simulink model "Hospital"  (R2020b)
settings: Solver=VariableStepAuto  StartTime=0.0  StopTime=10.0  RelTol=1e-3
libraries: dspstat3 x5
(part 1 of 2)
settings Model: Creator=Stefano  LastModifiedBy=stefanopanzieri
settings SFSimCC: CustomCodeUndefinedFunction=UseInterfaceOnly

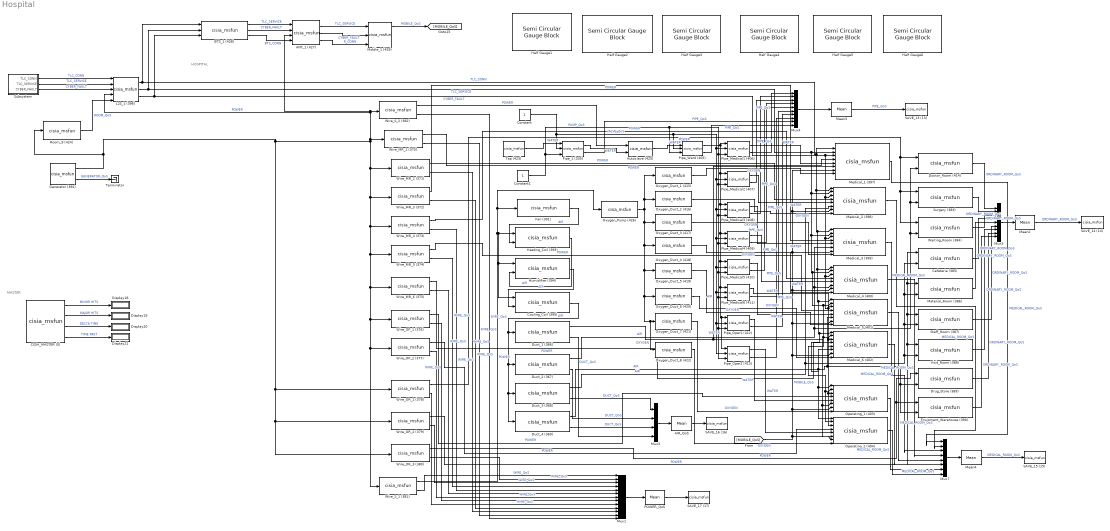
== system Hospital ==
  note: HOSPITAL
  note: MASTER
  AIR_QoS : dspstat3/Mean  run=off  InputProcessing=Columns as channels (frame based)  reset_popup=None  directionMode=Entire input  dimension=1  roiEnable=off  roiType=Rectangles  roiPortion=Entire ROI  roiOutput=Individual statistics for each ROI  roiFlag=off  roundingMode=Floor  overflowMode=off  outputDataTypeStr=Inherit: Same as accumulator  outputMin=[]  outputMax=[]  outputLastDataTypeStr=Inherit: Same as accumulator
  ANT_1 (427) : M-S-Function  FunctionName=cisia_msfun  Parameters=Parameter1, Parameter2, Parameter3, resources, Parameter10, codeupdate, step_received, step_computed, dynamic_computed, step_sended, id_entity, id_project, id_type, name_type, color  mask(S-function:msfcn_unit_delay){Parameter1='ANT_1', Parameter2=1, Parameter3='ORO', resources=, Parameter10=off, codeupdate=off, step_received=|, step_computed=, dynamic_computed=, step_sended=|, id_entity=427, id_project=6, id_type=55, name_type=CISCO_router, color=#EB7949}
      mask step_received=|
      | Connection=max(Connection_init,TLC_CONN);
      |
      | TLC_services=max(TLC_services_init,TLC_SERVICE);
      |
      |
      | Cyber_Fault=max(CYBER_FAULT, transpose([Dos_attack   MITM_attack  Port_Scan_Attack  Virus_Attack  BGP_hijacking]));
      |
      | % Vale 1 in presenza di fault
      | Conn_Fault=max([Dos_attack  Mechanical_Fault  1-POWER 1-ROOM_QoS] );
      |
      | Operative_Level=(1-Conn_Fault)*max(max(TLC_CONN),0.5);
      |
      |
      |
      | % Web Application Firewall and Enhanced application layer enrichment and protection
      mask step_sended=|
      | TLC_CONN=Connection*(1-Conn_Fault);
      | TLC_SERVICE=TLC_services*(1-Conn_Fault);
      | CYBER_FAULT=Cyber_Fault*(1-Conn_Fault);
      |
      | ROUTING_QoS=Operative_Level;
      mask prompts: Parameter1 "entity name"; Parameter2 "sampling time"; Parameter3 "project"; resources "input resources and state variables"; Parameter10 "Bring state variables to output"; codeupdate "update code from mask"
      mask help: This is a level-2 MATLAB file S-function which demonstrates CISIA entity
      mask DialogControl Container1 Prompt: All parameters
      mask Display: image('Icons/BTS_ANTENNA.png')
  Autoclave (425) : M-S-Function  FunctionName=cisia_msfun  Parameters=Parameter1, Parameter2, Parameter3, resources, Parameter10, codeupdate, step_received, step_computed, dynamic_computed, step_sended, id_entity, id_project, id_type, name_type, color  mask(S-function:msfcn_unit_delay){Parameter1='Autoclave', Parameter2=1, Parameter3='ORO', resources=, Parameter10=off, codeupdate=off, step_received=|, step_computed=, dynamic_computed=, step_sended=|, id_entity=425, id_project=6, id_type=33, name_type=Optical_Wire, color=#99CCFF}
      mask step_received=|
      | Connection=TLC_CONN;
      | TLC_services=TLC_SERVICE;
      | Cyber_Fault=CYBER_FAULT;
      |
      | Mechanical_Fault=max([Mechanical_Fault MECH_FAULT Mechanical_Fault_init]);
      |
      |
      | Operative_Level=1-Mechanical_Fault;
      mask step_sended=|
      | TLC_CONN=Connection*Operative_Level;
      | TLC_SERVICE=TLC_services*Operative_Level;
      | CYBER_FAULT=Cyber_Fault*Operative_Level;
      | MECH_FAULT=Mechanical_Fault;
      mask prompts: Parameter1 "entity name"; Parameter2 "sampling time"; Parameter3 "project"; resources "input resources and state variables"; Parameter10 "Bring state variables to output"; codeupdate "update code from mask"
      mask help: This is a level-2 MATLAB file S-function which demonstrates CISIA entity
      mask DialogControl Container1 Prompt: All parameters
      mask Display: disp('Autoclave')
  BTS_1 (428) : M-S-Function  FunctionName=cisia_msfun  Parameters=Parameter1, Parameter2, Parameter3, resources, Parameter10, codeupdate, step_received, step_computed, dynamic_computed, step_sended, id_entity, id_project, id_type, name_type, color  mask(S-function:msfcn_unit_delay){Parameter1='BTS_1', Parameter2=1, Parameter3='ORO', resources=, Parameter10=off, codeupdate=off, step_received=|, step_computed=, dynamic_computed=, step_sended=|, id_entity=428, id_project=6, id_type=54, name_type=CISCO_router, color=#EB7949}
      mask step_received=|
      | Connection=max(Connection_init,TLC_CONN);
      |
      | TLC_services=max(TLC_services_init,TLC_SERVICE);
      |
      |
      | Cyber_Fault=max(CYBER_FAULT, transpose([Dos_attack   MITM_attack  Port_Scan_Attack  Virus_Attack  BGP_hijacking]));
      |
      | % Vale 1 in presenza di fault
      | Conn_Fault=max([Dos_attack  Mechanical_Fault  1-POWER 1-ROOM_QoS] );
      |
      | Operative_Level=(1-Conn_Fault)*max(max(TLC_CONN),0.5);
      |
      |
      |
      | % Web Application Firewall and Enhanced application layer enrichment and protection
      mask step_sended=|
      | TLC_CONN=Connection*(1-Conn_Fault);
      | TLC_SERVICE=TLC_services*(1-Conn_Fault);
      | CYBER_FAULT=Cyber_Fault*(1-Conn_Fault);
      |
      | ROUTING_QoS=Operative_Level;
      mask prompts: Parameter1 "entity name"; Parameter2 "sampling time"; Parameter3 "project"; resources "input resources and state variables"; Parameter10 "Bring state variables to output"; codeupdate "update code from mask"
      mask help: This is a level-2 MATLAB file S-function which demonstrates CISIA entity
      mask DialogControl Container1 Prompt: All parameters
      mask Display: disp('BaseTransceiverStation')
  CISIA_MASTER (0) : M-S-Function  FunctionName=cisia_msfun  Parameters=Parameter1, Parameter2, Parameter3, resources, Parameter4, Parameter5, Parameter6, Parameter7, Parameter8, Parameter9  mask(S-function:msfcn_unit_delay){Parameter1='CISIA_MASTER', Parameter2=0.001, Parameter3='SistemiIoT', resources=off, Parameter4=on, Parameter5=off, Parameter6=off, Parameter7=off, Parameter8=1, Parameter9=off}
      mask prompts: Parameter1 "entity name"; Parameter2 "sampling time"; Parameter3 "project"; resources "Save status at each major hit"; Parameter4 "Show Operative Levels with colors"; Parameter5 "Load Entities from file"; Parameter6 "Load Start from Mask"; Parameter7 "Real Time"; Parameter8 "Real Time Hit (sec)"; Parameter9 "Skip saving"
      mask help: This is a level-2 MATLAB file S-function which demonstrates CISIA entity
      mask Display: disp('MASTER BLOCK')
  Cafeteria (385) : M-S-Function  FunctionName=cisia_msfun  Parameters=Parameter1, Parameter2, Parameter3, resources, Parameter10, codeupdate, step_received, step_computed, dynamic_computed, step_sended, id_entity, id_project, id_type, name_type, color  mask(S-function:msfcn_unit_delay){Parameter1='Cafeteria', Parameter2=1, Parameter3='ORO', resources=, Parameter10=off, codeupdate=off, step_received=|, step_computed=, dynamic_computed=, step_sended=|, id_entity=385, id_project=6, id_type=26, name_type=Optical_Wire, color=#99CCFF}
      mask step_received=|
      | Connection=TLC_CONN;
      | TLC_services=TLC_SERVICE;
      | Cyber_Fault=CYBER_FAULT;
      |
      | Mechanical_Fault=max([Mechanical_Fault MECH_FAULT Mechanical_Fault_init]);
      |
      |
      | Operative_Level=1-Mechanical_Fault;
      mask step_sended=|
      | TLC_CONN=Connection*Operative_Level;
      | TLC_SERVICE=TLC_services*Operative_Level;
      | CYBER_FAULT=Cyber_Fault*Operative_Level;
      | MECH_FAULT=Mechanical_Fault;
      mask prompts: Parameter1 "entity name"; Parameter2 "sampling time"; Parameter3 "project"; resources "input resources and state variables"; Parameter10 "Bring state variables to output"; codeupdate "update code from mask"
      mask help: This is a level-2 MATLAB file S-function which demonstrates CISIA entity
      mask DialogControl Container1 Prompt: All parameters
      mask Display: disp('Ordinary_Room')
  Constant : Constant
  Constant1 : Constant
  Cooling_Coil (395) : M-S-Function  FunctionName=cisia_msfun  Parameters=Parameter1, Parameter2, Parameter3, resources, Parameter10, codeupdate, step_received, step_computed, dynamic_computed, step_sended, id_entity, id_project, id_type, name_type, color  mask(S-function:msfcn_unit_delay){Parameter1='Cooling_Coil', Parameter2=1, Parameter3='ORO', resources=, Parameter10=off, codeupdate=off, step_received=|, step_computed=, dynamic_computed=, step_sended=|, id_entity=395, id_project=6, id_type=35, name_type=Optical_Wire, color=#99CCFF}
      mask step_received=|
      | Connection=TLC_CONN;
      | TLC_services=TLC_SERVICE;
      | Cyber_Fault=CYBER_FAULT;
      |
      | Mechanical_Fault=max([Mechanical_Fault MECH_FAULT Mechanical_Fault_init]);
      |
      |
      | Operative_Level=1-Mechanical_Fault;
      mask step_sended=|
      | TLC_CONN=Connection*Operative_Level;
      | TLC_SERVICE=TLC_services*Operative_Level;
      | CYBER_FAULT=Cyber_Fault*Operative_Level;
      | MECH_FAULT=Mechanical_Fault;
      mask prompts: Parameter1 "entity name"; Parameter2 "sampling time"; Parameter3 "project"; resources "input resources and state variables"; Parameter10 "Bring state variables to output"; codeupdate "update code from mask"
      mask help: This is a level-2 MATLAB file S-function which demonstrates CISIA entity
      mask DialogControl Container1 Prompt: All parameters
      mask Display: disp('Air_Conditioning_Element')
  Display{18..21} (4 alike) : Display
  Doctor_Room (414) : M-S-Function  FunctionName=cisia_msfun  Parameters=Parameter1, Parameter2, Parameter3, resources, Parameter10, codeupdate, step_received, step_computed, dynamic_computed, step_sended, id_entity, id_project, id_type, name_type, color  mask(S-function:msfcn_unit_delay){Parameter1='Doctor_Room', Parameter2=1, Parameter3='ORO', resources=, Parameter10=off, codeupdate=off, step_received=|, step_computed=, dynamic_computed=, step_sended=|, id_entity=414, id_project=6, id_type=26, name_type=Optical_Wire, color=#99CCFF}
      mask step_received=|
      | Connection=TLC_CONN;
      | TLC_services=TLC_SERVICE;
      | Cyber_Fault=CYBER_FAULT;
      |
      | Mechanical_Fault=max([Mechanical_Fault MECH_FAULT Mechanical_Fault_init]);
      |
      |
      | Operative_Level=1-Mechanical_Fault;
      mask step_sended=|
      | TLC_CONN=Connection*Operative_Level;
      | TLC_SERVICE=TLC_services*Operative_Level;
      | CYBER_FAULT=Cyber_Fault*Operative_Level;
      | MECH_FAULT=Mechanical_Fault;
      mask prompts: Parameter1 "entity name"; Parameter2 "sampling time"; Parameter3 "project"; resources "input resources and state variables"; Parameter10 "Bring state variables to output"; codeupdate "update code from mask"
      mask help: This is a level-2 MATLAB file S-function which demonstrates CISIA entity
      mask DialogControl Container1 Prompt: All parameters
      mask Display: disp('Ordinary_Room')
  Drug_Store (389) : M-S-Function  FunctionName=cisia_msfun  Parameters=Parameter1, Parameter2, Parameter3, resources, Parameter10, codeupdate, step_received, step_computed, dynamic_computed, step_sended, id_entity, id_project, id_type, name_type, color  mask(S-function:msfcn_unit_delay){Parameter1='Drug_Store', Parameter2=1, Parameter3='ORO', resources=, Parameter10=off, codeupdate=off, step_received=|, step_computed=, dynamic_computed=, step_sended=|, id_entity=389, id_project=6, id_type=26, name_type=Optical_Wire, color=#99CCFF}
      mask step_received=|
      | Connection=TLC_CONN;
      | TLC_services=TLC_SERVICE;
      | Cyber_Fault=CYBER_FAULT;
      |
      | Mechanical_Fault=max([Mechanical_Fault MECH_FAULT Mechanical_Fault_init]);
      |
      |
      | Operative_Level=1-Mechanical_Fault;
      mask step_sended=|
      | TLC_CONN=Connection*Operative_Level;
      | TLC_SERVICE=TLC_services*Operative_Level;
      | CYBER_FAULT=Cyber_Fault*Operative_Level;
      | MECH_FAULT=Mechanical_Fault;
      mask prompts: Parameter1 "entity name"; Parameter2 "sampling time"; Parameter3 "project"; resources "input resources and state variables"; Parameter10 "Bring state variables to output"; codeupdate "update code from mask"
      mask help: This is a level-2 MATLAB file S-function which demonstrates CISIA entity
      mask DialogControl Container1 Prompt: All parameters
      mask Display: disp('Ordinary_Room')
  Duct_1 (366) : M-S-Function  FunctionName=cisia_msfun  Parameters=Parameter1, Parameter2, Parameter3, resources, Parameter10, codeupdate, step_received, step_computed, dynamic_computed, step_sended, id_entity, id_project, id_type, name_type, color  mask(S-function:msfcn_unit_delay){Parameter1='Duct_1', Parameter2=1, Parameter3='ORO', resources=, Parameter10=off, codeupdate=off, step_received=|, step_computed=, dynamic_computed=, step_sended=|, id_entity=366, id_project=6, id_type=36, name_type=Optical_Wire, color=#99CCFF}
      mask step_received=|
      | Connection=TLC_CONN;
      | TLC_services=TLC_SERVICE;
      | Cyber_Fault=CYBER_FAULT;
      |
      | Mechanical_Fault=max([Mechanical_Fault MECH_FAULT Mechanical_Fault_init]);
      |
      |
      | Operative_Level=1-Mechanical_Fault;
      mask step_sended=|
      | TLC_CONN=Connection*Operative_Level;
      | TLC_SERVICE=TLC_services*Operative_Level;
      | CYBER_FAULT=Cyber_Fault*Operative_Level;
      | MECH_FAULT=Mechanical_Fault;
      mask prompts: Parameter1 "entity name"; Parameter2 "sampling time"; Parameter3 "project"; resources "input resources and state variables"; Parameter10 "Bring state variables to output"; codeupdate "update code from mask"
      mask help: This is a level-2 MATLAB file S-function which demonstrates CISIA entity
      mask DialogControl Container1 Prompt: All parameters
      mask Display: disp('Duct')
  Duct_2 (367) : M-S-Function  FunctionName=cisia_msfun  Parameters=Parameter1, Parameter2, Parameter3, resources, Parameter10, codeupdate, step_received, step_computed, dynamic_computed, step_sended, id_entity, id_project, id_type, name_type, color  mask(S-function:msfcn_unit_delay){Parameter1='Duct_2', Parameter2=1, Parameter3='ORO', resources=, Parameter10=off, codeupdate=off, step_received=|, step_computed=, dynamic_computed=, step_sended=|, id_entity=367, id_project=6, id_type=36, name_type=Optical_Wire, color=#99CCFF}
      mask step_received=|
      | Connection=TLC_CONN;
      | TLC_services=TLC_SERVICE;
      | Cyber_Fault=CYBER_FAULT;
      |
      | Mechanical_Fault=max([Mechanical_Fault MECH_FAULT Mechanical_Fault_init]);
      |
      |
      | Operative_Level=1-Mechanical_Fault;
      mask step_sended=|
      | TLC_CONN=Connection*Operative_Level;
      | TLC_SERVICE=TLC_services*Operative_Level;
      | CYBER_FAULT=Cyber_Fault*Operative_Level;
      | MECH_FAULT=Mechanical_Fault;
      mask prompts: Parameter1 "entity name"; Parameter2 "sampling time"; Parameter3 "project"; resources "input resources and state variables"; Parameter10 "Bring state variables to output"; codeupdate "update code from mask"
      mask help: This is a level-2 MATLAB file S-function which demonstrates CISIA entity
      mask DialogControl Container1 Prompt: All parameters
      mask Display: disp('Duct')
  Duct_3 (368) : M-S-Function  FunctionName=cisia_msfun  Parameters=Parameter1, Parameter2, Parameter3, resources, Parameter10, codeupdate, step_received, step_computed, dynamic_computed, step_sended, id_entity, id_project, id_type, name_type, color  mask(S-function:msfcn_unit_delay){Parameter1='Duct_3', Parameter2=1, Parameter3='ORO', resources=, Parameter10=off, codeupdate=off, step_received=|, step_computed=, dynamic_computed=, step_sended=|, id_entity=368, id_project=6, id_type=36, name_type=Optical_Wire, color=#99CCFF}
      mask step_received=|
      | Connection=TLC_CONN;
      | TLC_services=TLC_SERVICE;
      | Cyber_Fault=CYBER_FAULT;
      |
      | Mechanical_Fault=max([Mechanical_Fault MECH_FAULT Mechanical_Fault_init]);
      |
      |
      | Operative_Level=1-Mechanical_Fault;
      mask step_sended=|
      | TLC_CONN=Connection*Operative_Level;
      | TLC_SERVICE=TLC_services*Operative_Level;
      | CYBER_FAULT=Cyber_Fault*Operative_Level;
      | MECH_FAULT=Mechanical_Fault;
      mask prompts: Parameter1 "entity name"; Parameter2 "sampling time"; Parameter3 "project"; resources "input resources and state variables"; Parameter10 "Bring state variables to output"; codeupdate "update code from mask"
      mask help: This is a level-2 MATLAB file S-function which demonstrates CISIA entity
      mask DialogControl Container1 Prompt: All parameters
      mask Display: disp('Duct')
  Duct_4 (369) : M-S-Function  FunctionName=cisia_msfun  Parameters=Parameter1, Parameter2, Parameter3, resources, Parameter10, codeupdate, step_received, step_computed, dynamic_computed, step_sended, id_entity, id_project, id_type, name_type, color  mask(S-function:msfcn_unit_delay){Parameter1='Duct_4', Parameter2=1, Parameter3='ORO', resources=, Parameter10=off, codeupdate=off, step_received=|, step_computed=, dynamic_computed=, step_sended=|, id_entity=369, id_project=6, id_type=36, name_type=Optical_Wire, color=#99CCFF}
      mask step_received=|
      | Connection=TLC_CONN;
      | TLC_services=TLC_SERVICE;
      | Cyber_Fault=CYBER_FAULT;
      |
      | Mechanical_Fault=max([Mechanical_Fault MECH_FAULT Mechanical_Fault_init]);
      |
      |
      | Operative_Level=1-Mechanical_Fault;
      mask step_sended=|
      | TLC_CONN=Connection*Operative_Level;
      | TLC_SERVICE=TLC_services*Operative_Level;
      | CYBER_FAULT=Cyber_Fault*Operative_Level;
      | MECH_FAULT=Mechanical_Fault;
      mask prompts: Parameter1 "entity name"; Parameter2 "sampling time"; Parameter3 "project"; resources "input resources and state variables"; Parameter10 "Bring state variables to output"; codeupdate "update code from mask"
      mask help: This is a level-2 MATLAB file S-function which demonstrates CISIA entity
      mask DialogControl Container1 Prompt: All parameters
      mask Display: disp('Duct')
  Equipment_Warehouse (390) : M-S-Function  FunctionName=cisia_msfun  Parameters=Parameter1, Parameter2, Parameter3, resources, Parameter10, codeupdate, step_received, step_computed, dynamic_computed, step_sended, id_entity, id_project, id_type, name_type, color  mask(S-function:msfcn_unit_delay){Parameter1='Equipment_Warehouse', Parameter2=1, Parameter3='ORO', resources=, Parameter10=off, codeupdate=off, step_received=|, step_computed=, dynamic_computed=, step_sended=|, id_entity=390, id_project=6, id_type=26, name_type=Optical_Wire, color=#99CCFF}
      mask step_received=|
      | Connection=TLC_CONN;
      | TLC_services=TLC_SERVICE;
      | Cyber_Fault=CYBER_FAULT;
      |
      | Mechanical_Fault=max([Mechanical_Fault MECH_FAULT Mechanical_Fault_init]);
      |
      |
      | Operative_Level=1-Mechanical_Fault;
      mask step_sended=|
      | TLC_CONN=Connection*Operative_Level;
      | TLC_SERVICE=TLC_services*Operative_Level;
      | CYBER_FAULT=Cyber_Fault*Operative_Level;
      | MECH_FAULT=Mechanical_Fault;
      mask prompts: Parameter1 "entity name"; Parameter2 "sampling time"; Parameter3 "project"; resources "input resources and state variables"; Parameter10 "Bring state variables to output"; codeupdate "update code from mask"
      mask help: This is a level-2 MATLAB file S-function which demonstrates CISIA entity
      mask DialogControl Container1 Prompt: All parameters
      mask Display: disp('Ordinary_Room')
  Fan (391) : M-S-Function  FunctionName=cisia_msfun  Parameters=Parameter1, Parameter2, Parameter3, resources, Parameter10, codeupdate, step_received, step_computed, dynamic_computed, step_sended, id_entity, id_project, id_type, name_type, color  mask(S-function:msfcn_unit_delay){Parameter1='Fan', Parameter2=1, Parameter3='ORO', resources=, Parameter10=off, codeupdate=off, step_received=|, step_computed=, dynamic_computed=, step_sended=|, id_entity=391, id_project=6, id_type=34, name_type=Optical_Wire, color=#99CCFF}
      mask step_received=|
      | Connection=TLC_CONN;
      | TLC_services=TLC_SERVICE;
      | Cyber_Fault=CYBER_FAULT;
      |
      | Mechanical_Fault=max([Mechanical_Fault MECH_FAULT Mechanical_Fault_init]);
      |
      |
      | Operative_Level=1-Mechanical_Fault;
      mask step_sended=|
      | TLC_CONN=Connection*Operative_Level;
      | TLC_SERVICE=TLC_services*Operative_Level;
      | CYBER_FAULT=Cyber_Fault*Operative_Level;
      | MECH_FAULT=Mechanical_Fault;
      mask prompts: Parameter1 "entity name"; Parameter2 "sampling time"; Parameter3 "project"; resources "input resources and state variables"; Parameter10 "Bring state variables to output"; codeupdate "update code from mask"
      mask help: This is a level-2 MATLAB file S-function which demonstrates CISIA entity
      mask DialogControl Container1 Prompt: All parameters
      mask Display: disp('Fan')
  Generator (392) : M-S-Function  FunctionName=cisia_msfun  Parameters=Parameter1, Parameter2, Parameter3, resources, Parameter10, codeupdate, step_received, step_computed, dynamic_computed, step_sended, id_entity, id_project, id_type, name_type, color  mask(S-function:msfcn_unit_delay){Parameter1='Generator', Parameter2=1, Parameter3='ORO', resources=, Parameter10=off, codeupdate=off, step_received=|, step_computed=, dynamic_computed=, step_sended=|, id_entity=392, id_project=6, id_type=27, name_type=Optical_Wire, color=#99CCFF}
      mask step_received=|
      | Connection=TLC_CONN;
      | TLC_services=TLC_SERVICE;
      | Cyber_Fault=CYBER_FAULT;
      |
      | Mechanical_Fault=max([Mechanical_Fault MECH_FAULT Mechanical_Fault_init]);
      |
      |
      | Operative_Level=1-Mechanical_Fault;
      mask step_sended=|
      | TLC_CONN=Connection*Operative_Level;
      | TLC_SERVICE=TLC_services*Operative_Level;
      | CYBER_FAULT=Cyber_Fault*Operative_Level;
      | MECH_FAULT=Mechanical_Fault;
      mask prompts: Parameter1 "entity name"; Parameter2 "sampling time"; Parameter3 "project"; resources "input resources and state variables"; Parameter10 "Bring state variables to output"; codeupdate "update code from mask"
      mask help: This is a level-2 MATLAB file S-function which demonstrates CISIA entity
      mask DialogControl Container1 Prompt: All parameters
      mask Display: disp('Generator')
  Half Gauge{1..6} (6 alike) : SemiCircularGaugeBlock  ScaleMax=1
  Heating_Coil (393) : M-S-Function  FunctionName=cisia_msfun  Parameters=Parameter1, Parameter2, Parameter3, resources, Parameter10, codeupdate, step_received, step_computed, dynamic_computed, step_sended, id_entity, id_project, id_type, name_type, color  mask(S-function:msfcn_unit_delay){Parameter1='Heating_Coil', Parameter2=1, Parameter3='ORO', resources=, Parameter10=off, codeupdate=off, step_received=|, step_computed=, dynamic_computed=, step_sended=|, id_entity=393, id_project=6, id_type=35, name_type=Optical_Wire, color=#99CCFF}
      mask step_received=|
      | Connection=TLC_CONN;
      | TLC_services=TLC_SERVICE;
      | Cyber_Fault=CYBER_FAULT;
      |
      | Mechanical_Fault=max([Mechanical_Fault MECH_FAULT Mechanical_Fault_init]);
      |
      |
      | Operative_Level=1-Mechanical_Fault;
      mask step_sended=|
      | TLC_CONN=Connection*Operative_Level;
      | TLC_SERVICE=TLC_services*Operative_Level;
      | CYBER_FAULT=Cyber_Fault*Operative_Level;
      | MECH_FAULT=Mechanical_Fault;
      mask prompts: Parameter1 "entity name"; Parameter2 "sampling time"; Parameter3 "project"; resources "input resources and state variables"; Parameter10 "Bring state variables to output"; codeupdate "update code from mask"
      mask help: This is a level-2 MATLAB file S-function which demonstrates CISIA entity
      mask DialogControl Container1 Prompt: All parameters
      mask Display: disp('Air_Conditioning_Element')
  Humidifier (394) : M-S-Function  FunctionName=cisia_msfun  Parameters=Parameter1, Parameter2, Parameter3, resources, Parameter10, codeupdate, step_received, step_computed, dynamic_computed, step_sended, id_entity, id_project, id_type, name_type, color  mask(S-function:msfcn_unit_delay){Parameter1='Humidifier', Parameter2=1, Parameter3='ORO', resources=, Parameter10=off, codeupdate=off, step_received=|, step_computed=, dynamic_computed=, step_sended=|, id_entity=394, id_project=6, id_type=35, name_type=Optical_Wire, color=#99CCFF}
      mask step_received=|
      | Connection=TLC_CONN;
      | TLC_services=TLC_SERVICE;
      | Cyber_Fault=CYBER_FAULT;
      |
      | Mechanical_Fault=max([Mechanical_Fault MECH_FAULT Mechanical_Fault_init]);
      |
      |
      | Operative_Level=1-Mechanical_Fault;
      mask step_sended=|
      | TLC_CONN=Connection*Operative_Level;
      | TLC_SERVICE=TLC_services*Operative_Level;
      | CYBER_FAULT=Cyber_Fault*Operative_Level;
      | MECH_FAULT=Mechanical_Fault;
      mask prompts: Parameter1 "entity name"; Parameter2 "sampling time"; Parameter3 "project"; resources "input resources and state variables"; Parameter10 "Bring state variables to output"; codeupdate "update code from mask"
      mask help: This is a level-2 MATLAB file S-function which demonstrates CISIA entity
      mask DialogControl Container1 Prompt: All parameters
      mask Display: disp('Air_Conditioning_Element')
  L2S_1 (396) : M-S-Function  FunctionName=cisia_msfun  Parameters=Parameter1, Parameter2, Parameter3, resources, Parameter10, codeupdate, step_received, step_computed, dynamic_computed, step_sended, id_entity, id_project, id_type, name_type, color  mask(S-function:msfcn_unit_delay){Parameter1='L2S_1', Parameter2=1, Parameter3='ORO', resources=, Parameter10=off, codeupdate=off, step_received=|, step_computed=, dynamic_computed=, step_sended=|, id_entity=396, id_project=6, id_type=24, name_type=CISCO_router, color=#EB7949}
      mask step_received=|
      | Connection=max(Connection_init,TLC_CONN);
      |
      | TLC_services=max(TLC_services_init,TLC_SERVICE);
      |
      |
      | Cyber_Fault=max(CYBER_FAULT, transpose([Dos_attack   MITM_attack  Port_Scan_Attack  Virus_Attack  BGP_hijacking]));
      |
      | % Vale 1 in presenza di fault
      | Conn_Fault=max([Dos_attack  Mechanical_Fault  1-POWER 1-ROOM_QoS] );
      |
      | Operative_Level=(1-Conn_Fault)*max(max(TLC_CONN),0.5);
      |
      |
      |
      | % Web Application Firewall and Enhanced application layer enrichment and protection
      mask step_sended=|
      | TLC_CONN=Connection*(1-Conn_Fault);
      | TLC_SERVICE=TLC_services*(1-Conn_Fault);
      | CYBER_FAULT=Cyber_Fault*(1-Conn_Fault);
      |
      | ROUTING_QoS=Operative_Level;
      mask prompts: Parameter1 "entity name"; Parameter2 "sampling time"; Parameter3 "project"; resources "input resources and state variables"; Parameter10 "Bring state variables to output"; codeupdate "update code from mask"
      mask help: This is a level-2 MATLAB file S-function which demonstrates CISIA entity
      mask DialogControl Container1 Prompt: All parameters
      mask Display: image('Icons/Layer2Switch.png')
  Material_Room (386) : M-S-Function  FunctionName=cisia_msfun  Parameters=Parameter1, Parameter2, Parameter3, resources, Parameter10, codeupdate, step_received, step_computed, dynamic_computed, step_sended, id_entity, id_project, id_type, name_type, color  mask(S-function:msfcn_unit_delay){Parameter1='Material_Room', Parameter2=1, Parameter3='ORO', resources=, Parameter10=off, codeupdate=off, step_received=|, step_computed=, dynamic_computed=, step_sended=|, id_entity=386, id_project=6, id_type=26, name_type=Optical_Wire, color=#99CCFF}
      mask step_received=|
      | Connection=TLC_CONN;
      | TLC_services=TLC_SERVICE;
      | Cyber_Fault=CYBER_FAULT;
      |
      | Mechanical_Fault=max([Mechanical_Fault MECH_FAULT Mechanical_Fault_init]);
      |
      |
      | Operative_Level=1-Mechanical_Fault;
      mask step_sended=|
      | TLC_CONN=Connection*Operative_Level;
      | TLC_SERVICE=TLC_services*Operative_Level;
      | CYBER_FAULT=Cyber_Fault*Operative_Level;
      | MECH_FAULT=Mechanical_Fault;
      mask prompts: Parameter1 "entity name"; Parameter2 "sampling time"; Parameter3 "project"; resources "input resources and state variables"; Parameter10 "Bring state variables to output"; codeupdate "update code from mask"
      mask help: This is a level-2 MATLAB file S-function which demonstrates CISIA entity
      mask DialogControl Container1 Prompt: All parameters
      mask Display: disp('Ordinary_Room')
  Mean2 : dspstat3/Mean  run=off  InputProcessing=Columns as channels (frame based)  reset_popup=None  directionMode=Entire input  dimension=1  roiEnable=off  roiType=Rectangles  roiPortion=Entire ROI  roiOutput=Individual statistics for each ROI  roiFlag=off  roundingMode=Floor  overflowMode=off  outputDataTypeStr=Inherit: Same as accumulator  outputMin=[]  outputMax=[]  outputLastDataTypeStr=Inherit: Same as accumulator
  Mean3 : dspstat3/Mean  run=off  InputProcessing=Columns as channels (frame based)  reset_popup=None  directionMode=Entire input  dimension=1  roiEnable=off  roiType=Rectangles  roiPortion=Entire ROI  roiOutput=Individual statistics for each ROI  roiFlag=off  roundingMode=Floor  overflowMode=off  outputDataTypeStr=Inherit: Same as accumulator  outputMin=[]  outputMax=[]  outputLastDataTypeStr=Inherit: Same as accumulator
  Mean4 : dspstat3/Mean  run=off  InputProcessing=Columns as channels (frame based)  reset_popup=None  directionMode=Entire input  dimension=1  roiEnable=off  roiType=Rectangles  roiPortion=Entire ROI  roiOutput=Individual statistics for each ROI  roiFlag=off  roundingMode=Floor  overflowMode=off  outputDataTypeStr=Inherit: Same as accumulator  outputMin=[]  outputMax=[]  outputLastDataTypeStr=Inherit: Same as accumulator
  Medical_1 (397) : M-S-Function  FunctionName=cisia_msfun  Parameters=Parameter1, Parameter2, Parameter3, resources, Parameter10, codeupdate, step_received, step_computed, dynamic_computed, step_sended, id_entity, id_project, id_type, name_type, color  mask(S-function:msfcn_unit_delay){Parameter1='Medical_1', Parameter2=1, Parameter3='ORO', resources=, Parameter10=off, codeupdate=off, step_received=|, step_computed=, dynamic_computed=, step_sended=|, id_entity=397, id_project=6, id_type=25, name_type=Optical_Wire, color=#99CCFF}
      mask step_received=|
      | Connection=TLC_CONN;
      | TLC_services=TLC_SERVICE;
      | Cyber_Fault=CYBER_FAULT;
      |
      | Mechanical_Fault=max([Mechanical_Fault MECH_FAULT Mechanical_Fault_init]);
      |
      |
      | Operative_Level=1-Mechanical_Fault;
      mask step_sended=|
      | TLC_CONN=Connection*Operative_Level;
      | TLC_SERVICE=TLC_services*Operative_Level;
      | CYBER_FAULT=Cyber_Fault*Operative_Level;
      | MECH_FAULT=Mechanical_Fault;
      mask prompts: Parameter1 "entity name"; Parameter2 "sampling time"; Parameter3 "project"; resources "input resources and state variables"; Parameter10 "Bring state variables to output"; codeupdate "update code from mask"
      mask help: This is a level-2 MATLAB file S-function which demonstrates CISIA entity
      mask DialogControl Container1 Prompt: All parameters
      mask Display: disp('Medical_Room')
  Medical_2 (398) : M-S-Function  FunctionName=cisia_msfun  Parameters=Parameter1, Parameter2, Parameter3, resources, Parameter10, codeupdate, step_received, step_computed, dynamic_computed, step_sended, id_entity, id_project, id_type, name_type, color  mask(S-function:msfcn_unit_delay){Parameter1='Medical_2', Parameter2=1, Parameter3='ORO', resources=, Parameter10=off, codeupdate=off, step_received=|, step_computed=, dynamic_computed=, step_sended=|, id_entity=398, id_project=6, id_type=25, name_type=Optical_Wire, color=#99CCFF}
      mask step_received=|
      | Connection=TLC_CONN;
      | TLC_services=TLC_SERVICE;
      | Cyber_Fault=CYBER_FAULT;
      |
      | Mechanical_Fault=max([Mechanical_Fault MECH_FAULT Mechanical_Fault_init]);
      |
      |
      | Operative_Level=1-Mechanical_Fault;
      mask step_sended=|
      | TLC_CONN=Connection*Operative_Level;
      | TLC_SERVICE=TLC_services*Operative_Level;
      | CYBER_FAULT=Cyber_Fault*Operative_Level;
      | MECH_FAULT=Mechanical_Fault;
      mask prompts: Parameter1 "entity name"; Parameter2 "sampling time"; Parameter3 "project"; resources "input resources and state variables"; Parameter10 "Bring state variables to output"; codeupdate "update code from mask"
      mask help: This is a level-2 MATLAB file S-function which demonstrates CISIA entity
      mask DialogControl Container1 Prompt: All parameters
      mask Display: disp('Medical_Room')
  Medical_3 (399) : M-S-Function  FunctionName=cisia_msfun  Parameters=Parameter1, Parameter2, Parameter3, resources, Parameter10, codeupdate, step_received, step_computed, dynamic_computed, step_sended, id_entity, id_project, id_type, name_type, color  mask(S-function:msfcn_unit_delay){Parameter1='Medical_3', Parameter2=1, Parameter3='ORO', resources=, Parameter10=off, codeupdate=off, step_received=|, step_computed=, dynamic_computed=, step_sended=|, id_entity=399, id_project=6, id_type=25, name_type=Optical_Wire, color=#99CCFF}
      mask step_received=|
      | Connection=TLC_CONN;
      | TLC_services=TLC_SERVICE;
      | Cyber_Fault=CYBER_FAULT;
      |
      | Mechanical_Fault=max([Mechanical_Fault MECH_FAULT Mechanical_Fault_init]);
      |
      |
      | Operative_Level=1-Mechanical_Fault;
      mask step_sended=|
      | TLC_CONN=Connection*Operative_Level;
      | TLC_SERVICE=TLC_services*Operative_Level;
      | CYBER_FAULT=Cyber_Fault*Operative_Level;
      | MECH_FAULT=Mechanical_Fault;
      mask prompts: Parameter1 "entity name"; Parameter2 "sampling time"; Parameter3 "project"; resources "input resources and state variables"; Parameter10 "Bring state variables to output"; codeupdate "update code from mask"
      mask help: This is a level-2 MATLAB file S-function which demonstrates CISIA entity
      mask DialogControl Container1 Prompt: All parameters
      mask Display: disp('Medical_Room')
  Medical_4 (400) : M-S-Function  FunctionName=cisia_msfun  Parameters=Parameter1, Parameter2, Parameter3, resources, Parameter10, codeupdate, step_received, step_computed, dynamic_computed, step_sended, id_entity, id_project, id_type, name_type, color  mask(S-function:msfcn_unit_delay){Parameter1='Medical_4', Parameter2=1, Parameter3='ORO', resources=, Parameter10=off, codeupdate=off, step_received=|, step_computed=, dynamic_computed=, step_sended=|, id_entity=400, id_project=6, id_type=25, name_type=Optical_Wire, color=#99CCFF}
      mask step_received=|
      | Connection=TLC_CONN;
      | TLC_services=TLC_SERVICE;
      | Cyber_Fault=CYBER_FAULT;
      |
      | Mechanical_Fault=max([Mechanical_Fault MECH_FAULT Mechanical_Fault_init]);
      |
      |
      | Operative_Level=1-Mechanical_Fault;
      mask step_sended=|
      | TLC_CONN=Connection*Operative_Level;
      | TLC_SERVICE=TLC_services*Operative_Level;
      | CYBER_FAULT=Cyber_Fault*Operative_Level;
      | MECH_FAULT=Mechanical_Fault;
      mask prompts: Parameter1 "entity name"; Parameter2 "sampling time"; Parameter3 "project"; resources "input resources and state variables"; Parameter10 "Bring state variables to output"; codeupdate "update code from mask"
      mask help: This is a level-2 MATLAB file S-function which demonstrates CISIA entity
      mask DialogControl Container1 Prompt: All parameters
      mask Display: disp('Medical_Room')
  Medical_5 (401) : M-S-Function  FunctionName=cisia_msfun  Parameters=Parameter1, Parameter2, Parameter3, resources, Parameter10, codeupdate, step_received, step_computed, dynamic_computed, step_sended, id_entity, id_project, id_type, name_type, color  mask(S-function:msfcn_unit_delay){Parameter1='Medical_5', Parameter2=1, Parameter3='ORO', resources=, Parameter10=off, codeupdate=off, step_received=|, step_computed=, dynamic_computed=, step_sended=|, id_entity=401, id_project=6, id_type=25, name_type=Optical_Wire, color=#99CCFF}
      mask step_received=|
      | Connection=TLC_CONN;
      | TLC_services=TLC_SERVICE;
      | Cyber_Fault=CYBER_FAULT;
      |
      | Mechanical_Fault=max([Mechanical_Fault MECH_FAULT Mechanical_Fault_init]);
      |
      |
      | Operative_Level=1-Mechanical_Fault;
      mask step_sended=|
      | TLC_CONN=Connection*Operative_Level;
      | TLC_SERVICE=TLC_services*Operative_Level;
      | CYBER_FAULT=Cyber_Fault*Operative_Level;
      | MECH_FAULT=Mechanical_Fault;
      mask prompts: Parameter1 "entity name"; Parameter2 "sampling time"; Parameter3 "project"; resources "input resources and state variables"; Parameter10 "Bring state variables to output"; codeupdate "update code from mask"
      mask help: This is a level-2 MATLAB file S-function which demonstrates CISIA entity
      mask DialogControl Container1 Prompt: All parameters
      mask Display: disp('Medical_Room')
  Medical_6 (402) : M-S-Function  FunctionName=cisia_msfun  Parameters=Parameter1, Parameter2, Parameter3, resources, Parameter10, codeupdate, step_received, step_computed, dynamic_computed, step_sended, id_entity, id_project, id_type, name_type, color  mask(S-function:msfcn_unit_delay){Parameter1='Medical_6', Parameter2=1, Parameter3='ORO', resources=, Parameter10=off, codeupdate=off, step_received=|, step_computed=, dynamic_computed=, step_sended=|, id_entity=402, id_project=6, id_type=25, name_type=Optical_Wire, color=#99CCFF}
      mask step_received=|
      | Connection=TLC_CONN;
      | TLC_services=TLC_SERVICE;
      | Cyber_Fault=CYBER_FAULT;
      |
      | Mechanical_Fault=max([Mechanical_Fault MECH_FAULT Mechanical_Fault_init]);
      |
      |
      | Operative_Level=1-Mechanical_Fault;
      mask step_sended=|
      | TLC_CONN=Connection*Operative_Level;
      | TLC_SERVICE=TLC_services*Operative_Level;
      | CYBER_FAULT=Cyber_Fault*Operative_Level;
      | MECH_FAULT=Mechanical_Fault;
      mask prompts: Parameter1 "entity name"; Parameter2 "sampling time"; Parameter3 "project"; resources "input resources and state variables"; Parameter10 "Bring state variables to output"; codeupdate "update code from mask"
      mask help: This is a level-2 MATLAB file S-function which demonstrates CISIA entity
      mask DialogControl Container1 Prompt: All parameters
      mask Display: disp('Medical_Room')
  Mobile_1 (429) : M-S-Function  FunctionName=cisia_msfun  Parameters=Parameter1, Parameter2, Parameter3, resources, Parameter10, codeupdate, step_received, step_computed, dynamic_computed, step_sended, id_entity, id_project, id_type, name_type, color  mask(S-function:msfcn_unit_delay){Parameter1='Mobile_1', Parameter2=1, Parameter3='ORO', resources=, Parameter10=off, codeupdate=off, step_received=Operative_Level=R_CONN;, step_computed=, dynamic_computed=, step_sended=, id_entity=429, id_project=6, id_type=39, name_type=RU-DU_ANTENNA, color=#90DB5A}
      mask prompts: Parameter1 "entity name"; Parameter2 "sampling time"; Parameter3 "project"; resources "input resources and state variables"; Parameter10 "Bring state variables to output"; codeupdate "update code from mask"
      mask help: This is a level-2 MATLAB file S-function which demonstrates CISIA entity
      mask DialogControl Container1 Prompt: All parameters
      mask Display: image('Icons/MobileUnit.png')
  Mux1 : Mux  Inputs=13
  Mux3 : Mux
  Mux4 : Mux  Inputs=10
  Mux5 : Mux  Inputs=9
  Mux7 : Mux  Inputs=8
  Operating_1 (403) : M-S-Function  FunctionName=cisia_msfun  Parameters=Parameter1, Parameter2, Parameter3, resources, Parameter10, codeupdate, step_received, step_computed, dynamic_computed, step_sended, id_entity, id_project, id_type, name_type, color  mask(S-function:msfcn_unit_delay){Parameter1='Operating_1', Parameter2=1, Parameter3='ORO', resources=, Parameter10=off, codeupdate=off, step_received=|, step_computed=, dynamic_computed=, step_sended=|, id_entity=403, id_project=6, id_type=25, name_type=Optical_Wire, color=#99CCFF}
      mask step_received=|
      | Connection=TLC_CONN;
      | TLC_services=TLC_SERVICE;
      | Cyber_Fault=CYBER_FAULT;
      |
      | Mechanical_Fault=max([Mechanical_Fault MECH_FAULT Mechanical_Fault_init]);
      |
      |
      | Operative_Level=1-Mechanical_Fault;
      mask step_sended=|
      | TLC_CONN=Connection*Operative_Level;
      | TLC_SERVICE=TLC_services*Operative_Level;
      | CYBER_FAULT=Cyber_Fault*Operative_Level;
      | MECH_FAULT=Mechanical_Fault;
      mask prompts: Parameter1 "entity name"; Parameter2 "sampling time"; Parameter3 "project"; resources "input resources and state variables"; Parameter10 "Bring state variables to output"; codeupdate "update code from mask"
      mask help: This is a level-2 MATLAB file S-function which demonstrates CISIA entity
      mask DialogControl Container1 Prompt: All parameters
      mask Display: disp('Medical_Room')
  Operating_2 (404) : M-S-Function  FunctionName=cisia_msfun  Parameters=Parameter1, Parameter2, Parameter3, resources, Parameter10, codeupdate, step_received, step_computed, dynamic_computed, step_sended, id_entity, id_project, id_type, name_type, color  mask(S-function:msfcn_unit_delay){Parameter1='Operating_2', Parameter2=1, Parameter3='ORO', resources=, Parameter10=off, codeupdate=off, step_received=|, step_computed=, dynamic_computed=, step_sended=|, id_entity=404, id_project=6, id_type=25, name_type=Optical_Wire, color=#99CCFF}
      mask step_received=|
      | Connection=TLC_CONN;
      | TLC_services=TLC_SERVICE;
      | Cyber_Fault=CYBER_FAULT;
      |
      | Mechanical_Fault=max([Mechanical_Fault MECH_FAULT Mechanical_Fault_init]);
      |
      |
      | Operative_Level=1-Mechanical_Fault;
      mask step_sended=|
      | TLC_CONN=Connection*Operative_Level;
      | TLC_SERVICE=TLC_services*Operative_Level;
      | CYBER_FAULT=Cyber_Fault*Operative_Level;
      | MECH_FAULT=Mechanical_Fault;
      mask prompts: Parameter1 "entity name"; Parameter2 "sampling time"; Parameter3 "project"; resources "input resources and state variables"; Parameter10 "Bring state variables to output"; codeupdate "update code from mask"
      mask help: This is a level-2 MATLAB file S-function which demonstrates CISIA entity
      mask DialogControl Container1 Prompt: All parameters
      mask Display: disp('Medical_Room')
  Oxygen_Duct_1 (415) : M-S-Function  FunctionName=cisia_msfun  Parameters=Parameter1, Parameter2, Parameter3, resources, Parameter10, codeupdate, step_received, step_computed, dynamic_computed, step_sended, id_entity, id_project, id_type, name_type, color  mask(S-function:msfcn_unit_delay){Parameter1='Oxygen_Duct_1', Parameter2=1, Parameter3='ORO', resources=, Parameter10=off, codeupdate=off, step_received=|, step_computed=, dynamic_computed=, step_sended=|, id_entity=415, id_project=6, id_type=57, name_type=Optical_Wire, color=#99CCFF}
      mask step_received=|
      | Connection=TLC_CONN;
      | TLC_services=TLC_SERVICE;
      | Cyber_Fault=CYBER_FAULT;
      |
      | Mechanical_Fault=max([Mechanical_Fault MECH_FAULT Mechanical_Fault_init]);
      |
      |
      | Operative_Level=1-Mechanical_Fault;
      mask step_sended=|
      | TLC_CONN=Connection*Operative_Level;
      | TLC_SERVICE=TLC_services*Operative_Level;
      | CYBER_FAULT=Cyber_Fault*Operative_Level;
      | MECH_FAULT=Mechanical_Fault;
      mask prompts: Parameter1 "entity name"; Parameter2 "sampling time"; Parameter3 "project"; resources "input resources and state variables"; Parameter10 "Bring state variables to output"; codeupdate "update code from mask"
      mask help: This is a level-2 MATLAB file S-function which demonstrates CISIA entity
      mask DialogControl Container1 Prompt: All parameters
      mask Display: disp('OXYGEN_Duct')
  Oxygen_Duct_2 (416) : M-S-Function  FunctionName=cisia_msfun  Parameters=Parameter1, Parameter2, Parameter3, resources, Parameter10, codeupdate, step_received, step_computed, dynamic_computed, step_sended, id_entity, id_project, id_type, name_type, color  mask(S-function:msfcn_unit_delay){Parameter1='Oxygen_Duct_2', Parameter2=1, Parameter3='ORO', resources=, Parameter10=off, codeupdate=off, step_received=|, step_computed=, dynamic_computed=, step_sended=|, id_entity=416, id_project=6, id_type=57, name_type=Optical_Wire, color=#99CCFF}
      mask step_received=|
      | Connection=TLC_CONN;
      | TLC_services=TLC_SERVICE;
      | Cyber_Fault=CYBER_FAULT;
      |
      | Mechanical_Fault=max([Mechanical_Fault MECH_FAULT Mechanical_Fault_init]);
      |
      |
      | Operative_Level=1-Mechanical_Fault;
      mask step_sended=|
      | TLC_CONN=Connection*Operative_Level;
      | TLC_SERVICE=TLC_services*Operative_Level;
      | CYBER_FAULT=Cyber_Fault*Operative_Level;
      | MECH_FAULT=Mechanical_Fault;
      mask prompts: Parameter1 "entity name"; Parameter2 "sampling time"; Parameter3 "project"; resources "input resources and state variables"; Parameter10 "Bring state variables to output"; codeupdate "update code from mask"
      mask help: This is a level-2 MATLAB file S-function which demonstrates CISIA entity
      mask DialogControl Container1 Prompt: All parameters
      mask Display: disp('OXYGEN_Duct')
  Oxygen_Duct_3 (417) : M-S-Function  FunctionName=cisia_msfun  Parameters=Parameter1, Parameter2, Parameter3, resources, Parameter10, codeupdate, step_received, step_computed, dynamic_computed, step_sended, id_entity, id_project, id_type, name_type, color  mask(S-function:msfcn_unit_delay){Parameter1='Oxygen_Duct_3', Parameter2=1, Parameter3='ORO', resources=, Parameter10=off, codeupdate=off, step_received=|, step_computed=, dynamic_computed=, step_sended=|, id_entity=417, id_project=6, id_type=57, name_type=Optical_Wire, color=#99CCFF}
      mask step_received=|
      | Connection=TLC_CONN;
      | TLC_services=TLC_SERVICE;
      | Cyber_Fault=CYBER_FAULT;
      |
      | Mechanical_Fault=max([Mechanical_Fault MECH_FAULT Mechanical_Fault_init]);
      |
      |
      | Operative_Level=1-Mechanical_Fault;
      mask step_sended=|
      | TLC_CONN=Connection*Operative_Level;
      | TLC_SERVICE=TLC_services*Operative_Level;
      | CYBER_FAULT=Cyber_Fault*Operative_Level;
      | MECH_FAULT=Mechanical_Fault;
      mask prompts: Parameter1 "entity name"; Parameter2 "sampling time"; Parameter3 "project"; resources "input resources and state variables"; Parameter10 "Bring state variables to output"; codeupdate "update code from mask"
      mask help: This is a level-2 MATLAB file S-function which demonstrates CISIA entity
      mask DialogControl Container1 Prompt: All parameters
      mask Display: disp('OXYGEN_Duct')
  Oxygen_Duct_4 (418) : M-S-Function  FunctionName=cisia_msfun  Parameters=Parameter1, Parameter2, Parameter3, resources, Parameter10, codeupdate, step_received, step_computed, dynamic_computed, step_sended, id_entity, id_project, id_type, name_type, color  mask(S-function:msfcn_unit_delay){Parameter1='Oxygen_Duct_4', Parameter2=1, Parameter3='ORO', resources=, Parameter10=off, codeupdate=off, step_received=|, step_computed=, dynamic_computed=, step_sended=|, id_entity=418, id_project=6, id_type=57, name_type=Optical_Wire, color=#99CCFF}
      mask step_received=|
      | Connection=TLC_CONN;
      | TLC_services=TLC_SERVICE;
      | Cyber_Fault=CYBER_FAULT;
      |
      | Mechanical_Fault=max([Mechanical_Fault MECH_FAULT Mechanical_Fault_init]);
      |
      |
      | Operative_Level=1-Mechanical_Fault;
      mask step_sended=|
      | TLC_CONN=Connection*Operative_Level;
      | TLC_SERVICE=TLC_services*Operative_Level;
      | CYBER_FAULT=Cyber_Fault*Operative_Level;
      | MECH_FAULT=Mechanical_Fault;
      mask prompts: Parameter1 "entity name"; Parameter2 "sampling time"; Parameter3 "project"; resources "input resources and state variables"; Parameter10 "Bring state variables to output"; codeupdate "update code from mask"
      mask help: This is a level-2 MATLAB file S-function which demonstrates CISIA entity
      mask DialogControl Container1 Prompt: All parameters
      mask Display: disp('OXYGEN_Duct')
  Oxygen_Duct_5 (419) : M-S-Function  FunctionName=cisia_msfun  Parameters=Parameter1, Parameter2, Parameter3, resources, Parameter10, codeupdate, step_received, step_computed, dynamic_computed, step_sended, id_entity, id_project, id_type, name_type, color  mask(S-function:msfcn_unit_delay){Parameter1='Oxygen_Duct_5', Parameter2=1, Parameter3='ORO', resources=, Parameter10=off, codeupdate=off, step_received=|, step_computed=, dynamic_computed=, step_sended=|, id_entity=419, id_project=6, id_type=57, name_type=Optical_Wire, color=#99CCFF}
      mask step_received=|
      | Connection=TLC_CONN;
      | TLC_services=TLC_SERVICE;
      | Cyber_Fault=CYBER_FAULT;
      |
      | Mechanical_Fault=max([Mechanical_Fault MECH_FAULT Mechanical_Fault_init]);
      |
      |
      | Operative_Level=1-Mechanical_Fault;
      mask step_sended=|
      | TLC_CONN=Connection*Operative_Level;
      | TLC_SERVICE=TLC_services*Operative_Level;
      | CYBER_FAULT=Cyber_Fault*Operative_Level;
      | MECH_FAULT=Mechanical_Fault;
      mask prompts: Parameter1 "entity name"; Parameter2 "sampling time"; Parameter3 "project"; resources "input resources and state variables"; Parameter10 "Bring state variables to output"; codeupdate "update code from mask"
      mask help: This is a level-2 MATLAB file S-function which demonstrates CISIA entity
      mask DialogControl Container1 Prompt: All parameters
      mask Display: disp('OXYGEN_Duct')
  Oxygen_Duct_6 (420) : M-S-Function  FunctionName=cisia_msfun  Parameters=Parameter1, Parameter2, Parameter3, resources, Parameter10, codeupdate, step_received, step_computed, dynamic_computed, step_sended, id_entity, id_project, id_type, name_type, color  mask(S-function:msfcn_unit_delay){Parameter1='Oxygen_Duct_6', Parameter2=1, Parameter3='ORO', resources=, Parameter10=off, codeupdate=off, step_received=|, step_computed=, dynamic_computed=, step_sended=|, id_entity=420, id_project=6, id_type=57, name_type=Optical_Wire, color=#99CCFF}
      mask step_received=|
      | Connection=TLC_CONN;
      | TLC_services=TLC_SERVICE;
      | Cyber_Fault=CYBER_FAULT;
      |
      | Mechanical_Fault=max([Mechanical_Fault MECH_FAULT Mechanical_Fault_init]);
      |
      |
      | Operative_Level=1-Mechanical_Fault;
      mask step_sended=|
      | TLC_CONN=Connection*Operative_Level;
      | TLC_SERVICE=TLC_services*Operative_Level;
      | CYBER_FAULT=Cyber_Fault*Operative_Level;
      | MECH_FAULT=Mechanical_Fault;
      mask prompts: Parameter1 "entity name"; Parameter2 "sampling time"; Parameter3 "project"; resources "input resources and state variables"; Parameter10 "Bring state variables to output"; codeupdate "update code from mask"
      mask help: This is a level-2 MATLAB file S-function which demonstrates CISIA entity
      mask DialogControl Container1 Prompt: All parameters
      mask Display: disp('OXYGEN_Duct')
  Oxygen_Duct_7 (421) : M-S-Function  FunctionName=cisia_msfun  Parameters=Parameter1, Parameter2, Parameter3, resources, Parameter10, codeupdate, step_received, step_computed, dynamic_computed, step_sended, id_entity, id_project, id_type, name_type, color  mask(S-function:msfcn_unit_delay){Parameter1='Oxygen_Duct_7', Parameter2=1, Parameter3='ORO', resources=, Parameter10=off, codeupdate=off, step_received=|, step_computed=, dynamic_computed=, step_sended=|, id_entity=421, id_project=6, id_type=57, name_type=Optical_Wire, color=#99CCFF}
      mask step_received=|
      | Connection=TLC_CONN;
      | TLC_services=TLC_SERVICE;
      | Cyber_Fault=CYBER_FAULT;
      |
      | Mechanical_Fault=max([Mechanical_Fault MECH_FAULT Mechanical_Fault_init]);
      |
      |
      | Operative_Level=1-Mechanical_Fault;
      mask step_sended=|
      | TLC_CONN=Connection*Operative_Level;
      | TLC_SERVICE=TLC_services*Operative_Level;
      | CYBER_FAULT=Cyber_Fault*Operative_Level;
      | MECH_FAULT=Mechanical_Fault;
      mask prompts: Parameter1 "entity name"; Parameter2 "sampling time"; Parameter3 "project"; resources "input resources and state variables"; Parameter10 "Bring state variables to output"; codeupdate "update code from mask"
      mask help: This is a level-2 MATLAB file S-function which demonstrates CISIA entity
      mask DialogControl Container1 Prompt: All parameters
      mask Display: disp('OXYGEN_Duct')
  Oxygen_Duct_8 (422) : M-S-Function  FunctionName=cisia_msfun  Parameters=Parameter1, Parameter2, Parameter3, resources, Parameter10, codeupdate, step_received, step_computed, dynamic_computed, step_sended, id_entity, id_project, id_type, name_type, color  mask(S-function:msfcn_unit_delay){Parameter1='Oxygen_Duct_8', Parameter2=1, Parameter3='ORO', resources=, Parameter10=off, codeupdate=off, step_received=|, step_computed=, dynamic_computed=, step_sended=|, id_entity=422, id_project=6, id_type=57, name_type=Optical_Wire, color=#99CCFF}
      mask step_received=|
      | Connection=TLC_CONN;
      | TLC_services=TLC_SERVICE;
      | Cyber_Fault=CYBER_FAULT;
      |
      | Mechanical_Fault=max([Mechanical_Fault MECH_FAULT Mechanical_Fault_init]);
      |
      |
      | Operative_Level=1-Mechanical_Fault;
      mask step_sended=|
      | TLC_CONN=Connection*Operative_Level;
      | TLC_SERVICE=TLC_services*Operative_Level;
      | CYBER_FAULT=Cyber_Fault*Operative_Level;
      | MECH_FAULT=Mechanical_Fault;
      mask prompts: Parameter1 "entity name"; Parameter2 "sampling time"; Parameter3 "project"; resources "input resources and state variables"; Parameter10 "Bring state variables to output"; codeupdate "update code from mask"
      mask help: This is a level-2 MATLAB file S-function which demonstrates CISIA entity
      mask DialogControl Container1 Prompt: All parameters
      mask Display: disp('OXYGEN_Duct')
  Oxygen_Pump (426) : M-S-Function  FunctionName=cisia_msfun  Parameters=Parameter1, Parameter2, Parameter3, resources, Parameter10, codeupdate, step_received, step_computed, dynamic_computed, step_sended, id_entity, id_project, id_type, name_type, color  mask(S-function:msfcn_unit_delay){Parameter1='Oxygen_Pump', Parameter2=1, Parameter3='ORO', resources=, Parameter10=off, codeupdate=off, step_received=|, step_computed=, dynamic_computed=, step_sended=|, id_entity=426, id_project=6, id_type=56, name_type=Optical_Wire, color=#99CCFF}
      mask step_received=|
      | Connection=TLC_CONN;
      | TLC_services=TLC_SERVICE;
      | Cyber_Fault=CYBER_FAULT;
      |
      | Mechanical_Fault=max([Mechanical_Fault MECH_FAULT Mechanical_Fault_init]);
      |
      |
      | Operative_Level=1-Mechanical_Fault;
      mask step_sended=|
      | TLC_CONN=Connection*Operative_Level;
      | TLC_SERVICE=TLC_services*Operative_Level;
      | CYBER_FAULT=Cyber_Fault*Operative_Level;
      | MECH_FAULT=Mechanical_Fault;
      mask prompts: Parameter1 "entity name"; Parameter2 "sampling time"; Parameter3 "project"; resources "input resources and state variables"; Parameter10 "Bring state variables to output"; codeupdate "update code from mask"
      mask help: This is a level-2 MATLAB file S-function which demonstrates CISIA entity
      mask DialogControl Container1 Prompt: All parameters
      mask Display: disp('OXYGEN_Element')
  POWER_QoS : dspstat3/Mean  run=off  InputProcessing=Columns as channels (frame based)  reset_popup=None  directionMode=Entire input  dimension=1  roiEnable=off  roiType=Rectangles  roiPortion=Entire ROI  roiOutput=Individual statistics for each ROI  roiFlag=off  roundingMode=Floor  overflowMode=off  outputDataTypeStr=Inherit: Same as accumulator  outputMin=[]  outputMax=[]  outputLastDataTypeStr=Inherit: Same as accumulator
  Pipe_1 (335) : M-S-Function  FunctionName=cisia_msfun  Parameters=Parameter1, Parameter2, Parameter3, resources, Parameter10, codeupdate, step_received, step_computed, dynamic_computed, step_sended, id_entity, id_project, id_type, name_type, color  mask(S-function:msfcn_unit_delay){Parameter1='Pipe_1', Parameter2=1, Parameter3='ORO', resources=, Parameter10=off, codeupdate=off, step_received=|, step_computed=, dynamic_computed=, step_sended=|, id_entity=335, id_project=6, id_type=84, name_type=Optical_Wire, color=#99CCFF}
      mask step_received=|
      | Connection=TLC_CONN;
      | TLC_services=TLC_SERVICE;
      | Cyber_Fault=CYBER_FAULT;
      |
      | Mechanical_Fault=max([Mechanical_Fault MECH_FAULT Mechanical_Fault_init]);
      |
      |
      | Operative_Level=1-Mechanical_Fault;
      mask step_sended=|
      | TLC_CONN=Connection*Operative_Level;
      | TLC_SERVICE=TLC_services*Operative_Level;
      | CYBER_FAULT=Cyber_Fault*Operative_Level;
      | MECH_FAULT=Mechanical_Fault;
      mask prompts: Parameter1 "entity name"; Parameter2 "sampling time"; Parameter3 "project"; resources "input resources and state variables"; Parameter10 "Bring state variables to output"; codeupdate "update code from mask"
      mask help: This is a level-2 MATLAB file S-function which demonstrates CISIA entity
      mask DialogControl Container1 Prompt: All parameters
      mask Display: image('Icons/Pipe.png')
  Pipe_Medical1 (406) : M-S-Function  FunctionName=cisia_msfun  Parameters=Parameter1, Parameter2, Parameter3, resources, Parameter10, codeupdate, step_received, step_computed, dynamic_computed, step_sended, id_entity, id_project, id_type, name_type, color  mask(S-function:msfcn_unit_delay){Parameter1='Pipe_Medical1', Parameter2=1, Parameter3='ORO', resources=, Parameter10=off, codeupdate=off, step_received=|, step_computed=, dynamic_computed=, step_sended=|, id_entity=406, id_project=6, id_type=84, name_type=Optical_Wire, color=#99CCFF}
      mask step_received=|
      | Connection=TLC_CONN;
      | TLC_services=TLC_SERVICE;
      | Cyber_Fault=CYBER_FAULT;
      |
      | Mechanical_Fault=max([Mechanical_Fault MECH_FAULT Mechanical_Fault_init]);
      |
      |
      | Operative_Level=1-Mechanical_Fault;
      mask step_sended=|
      | TLC_CONN=Connection*Operative_Level;
      | TLC_SERVICE=TLC_services*Operative_Level;
      | CYBER_FAULT=Cyber_Fault*Operative_Level;
      | MECH_FAULT=Mechanical_Fault;
      mask prompts: Parameter1 "entity name"; Parameter2 "sampling time"; Parameter3 "project"; resources "input resources and state variables"; Parameter10 "Bring state variables to output"; codeupdate "update code from mask"
      mask help: This is a level-2 MATLAB file S-function which demonstrates CISIA entity
      mask DialogControl Container1 Prompt: All parameters
      mask Display: image('Icons/Pipe.png')
  Pipe_Medical2 (407) : M-S-Function  FunctionName=cisia_msfun  Parameters=Parameter1, Parameter2, Parameter3, resources, Parameter10, codeupdate, step_received, step_computed, dynamic_computed, step_sended, id_entity, id_project, id_type, name_type, color  mask(S-function:msfcn_unit_delay){Parameter1='Pipe_Medical2', Parameter2=1, Parameter3='ORO', resources=, Parameter10=off, codeupdate=off, step_received=|, step_computed=, dynamic_computed=, step_sended=|, id_entity=407, id_project=6, id_type=84, name_type=Optical_Wire, color=#99CCFF}
      mask step_received=|
      | Connection=TLC_CONN;
      | TLC_services=TLC_SERVICE;
      | Cyber_Fault=CYBER_FAULT;
      |
      | Mechanical_Fault=max([Mechanical_Fault MECH_FAULT Mechanical_Fault_init]);
      |
      |
      | Operative_Level=1-Mechanical_Fault;
      mask step_sended=|
      | TLC_CONN=Connection*Operative_Level;
      | TLC_SERVICE=TLC_services*Operative_Level;
      | CYBER_FAULT=Cyber_Fault*Operative_Level;
      | MECH_FAULT=Mechanical_Fault;
      mask prompts: Parameter1 "entity name"; Parameter2 "sampling time"; Parameter3 "project"; resources "input resources and state variables"; Parameter10 "Bring state variables to output"; codeupdate "update code from mask"
      mask help: This is a level-2 MATLAB file S-function which demonstrates CISIA entity
      mask DialogControl Container1 Prompt: All parameters
      mask Display: image('Icons/Pipe.png')
  Pipe_Medical3 (408) : M-S-Function  FunctionName=cisia_msfun  Parameters=Parameter1, Parameter2, Parameter3, resources, Parameter10, codeupdate, step_received, step_computed, dynamic_computed, step_sended, id_entity, id_project, id_type, name_type, color  mask(S-function:msfcn_unit_delay){Parameter1='Pipe_Medical3', Parameter2=1, Parameter3='ORO', resources=, Parameter10=off, codeupdate=off, step_received=|, step_computed=, dynamic_computed=, step_sended=|, id_entity=408, id_project=6, id_type=84, name_type=Optical_Wire, color=#99CCFF}
      mask step_received=|
      | Connection=TLC_CONN;
      | TLC_services=TLC_SERVICE;
      | Cyber_Fault=CYBER_FAULT;
      |
      | Mechanical_Fault=max([Mechanical_Fault MECH_FAULT Mechanical_Fault_init]);
      |
      |
      | Operative_Level=1-Mechanical_Fault;
      mask step_sended=|
      | TLC_CONN=Connection*Operative_Level;
      | TLC_SERVICE=TLC_services*Operative_Level;
      | CYBER_FAULT=Cyber_Fault*Operative_Level;
      | MECH_FAULT=Mechanical_Fault;
      mask prompts: Parameter1 "entity name"; Parameter2 "sampling time"; Parameter3 "project"; resources "input resources and state variables"; Parameter10 "Bring state variables to output"; codeupdate "update code from mask"
      mask help: This is a level-2 MATLAB file S-function which demonstrates CISIA entity
      mask DialogControl Container1 Prompt: All parameters
      mask Display: image('Icons/Pipe.png')
  Pipe_Medical4 (409) : M-S-Function  FunctionName=cisia_msfun  Parameters=Parameter1, Parameter2, Parameter3, resources, Parameter10, codeupdate, step_received, step_computed, dynamic_computed, step_sended, id_entity, id_project, id_type, name_type, color  mask(S-function:msfcn_unit_delay){Parameter1='Pipe_Medical4', Parameter2=1, Parameter3='ORO', resources=, Parameter10=off, codeupdate=off, step_received=|, step_computed=, dynamic_computed=, step_sended=|, id_entity=409, id_project=6, id_type=84, name_type=Optical_Wire, color=#99CCFF}
      mask step_received=|
      | Connection=TLC_CONN;
      | TLC_services=TLC_SERVICE;
      | Cyber_Fault=CYBER_FAULT;
      |
      | Mechanical_Fault=max([Mechanical_Fault MECH_FAULT Mechanical_Fault_init]);
      |
      |
      | Operative_Level=1-Mechanical_Fault;
      mask step_sended=|
      | TLC_CONN=Connection*Operative_Level;
      | TLC_SERVICE=TLC_services*Operative_Level;
      | CYBER_FAULT=Cyber_Fault*Operative_Level;
      | MECH_FAULT=Mechanical_Fault;
      mask prompts: Parameter1 "entity name"; Parameter2 "sampling time"; Parameter3 "project"; resources "input resources and state variables"; Parameter10 "Bring state variables to output"; codeupdate "update code from mask"
      mask help: This is a level-2 MATLAB file S-function which demonstrates CISIA entity
      mask DialogControl Container1 Prompt: All parameters
      mask Display: image('Icons/Pipe.png')
  Pipe_Medical5 (410) : M-S-Function  FunctionName=cisia_msfun  Parameters=Parameter1, Parameter2, Parameter3, resources, Parameter10, codeupdate, step_received, step_computed, dynamic_computed, step_sended, id_entity, id_project, id_type, name_type, color  mask(S-function:msfcn_unit_delay){Parameter1='Pipe_Medical5', Parameter2=1, Parameter3='ORO', resources=, Parameter10=off, codeupdate=off, step_received=|, step_computed=, dynamic_computed=, step_sended=|, id_entity=410, id_project=6, id_type=84, name_type=Optical_Wire, color=#99CCFF}
      mask step_received=|
      | Connection=TLC_CONN;
      | TLC_services=TLC_SERVICE;
      | Cyber_Fault=CYBER_FAULT;
      |
      | Mechanical_Fault=max([Mechanical_Fault MECH_FAULT Mechanical_Fault_init]);
      |
      |
      | Operative_Level=1-Mechanical_Fault;
      mask step_sended=|
      | TLC_CONN=Connection*Operative_Level;
      | TLC_SERVICE=TLC_services*Operative_Level;
      | CYBER_FAULT=Cyber_Fault*Operative_Level;
      | MECH_FAULT=Mechanical_Fault;
      mask prompts: Parameter1 "entity name"; Parameter2 "sampling time"; Parameter3 "project"; resources "input resources and state variables"; Parameter10 "Bring state variables to output"; codeupdate "update code from mask"
      mask help: This is a level-2 MATLAB file S-function which demonstrates CISIA entity
      mask DialogControl Container1 Prompt: All parameters
      mask Display: image('Icons/Pipe.png')
  Pipe_Medical6 (411) : M-S-Function  FunctionName=cisia_msfun  Parameters=Parameter1, Parameter2, Parameter3, resources, Parameter10, codeupdate, step_received, step_computed, dynamic_computed, step_sended, id_entity, id_project, id_type, name_type, color  mask(S-function:msfcn_unit_delay){Parameter1='Pipe_Medical6', Parameter2=1, Parameter3='ORO', resources=, Parameter10=off, codeupdate=off, step_received=|, step_computed=, dynamic_computed=, step_sended=|, id_entity=411, id_project=6, id_type=84, name_type=Optical_Wire, color=#99CCFF}
      mask step_received=|
      | Connection=TLC_CONN;
      | TLC_services=TLC_SERVICE;
      | Cyber_Fault=CYBER_FAULT;
      |
      | Mechanical_Fault=max([Mechanical_Fault MECH_FAULT Mechanical_Fault_init]);
      |
      |
      | Operative_Level=1-Mechanical_Fault;
      mask step_sended=|
      | TLC_CONN=Connection*Operative_Level;
      | TLC_SERVICE=TLC_services*Operative_Level;
      | CYBER_FAULT=Cyber_Fault*Operative_Level;
      | MECH_FAULT=Mechanical_Fault;
      mask prompts: Parameter1 "entity name"; Parameter2 "sampling time"; Parameter3 "project"; resources "input resources and state variables"; Parameter10 "Bring state variables to output"; codeupdate "update code from mask"
      mask help: This is a level-2 MATLAB file S-function which demonstrates CISIA entity
      mask DialogControl Container1 Prompt: All parameters
      mask Display: image('Icons/Pipe.png')
  Pipe_Oper1 (412) : M-S-Function  FunctionName=cisia_msfun  Parameters=Parameter1, Parameter2, Parameter3, resources, Parameter10, codeupdate, step_received, step_computed, dynamic_computed, step_sended, id_entity, id_project, id_type, name_type, color  mask(S-function:msfcn_unit_delay){Parameter1='Pipe_Oper1', Parameter2=1, Parameter3='ORO', resources=, Parameter10=off, codeupdate=off, step_received=|, step_computed=, dynamic_computed=, step_sended=|, id_entity=412, id_project=6, id_type=84, name_type=Optical_Wire, color=#99CCFF}
      mask step_received=|
      | Connection=TLC_CONN;
      | TLC_services=TLC_SERVICE;
      | Cyber_Fault=CYBER_FAULT;
      |
      | Mechanical_Fault=max([Mechanical_Fault MECH_FAULT Mechanical_Fault_init]);
      |
      |
      | Operative_Level=1-Mechanical_Fault;
      mask step_sended=|
      | TLC_CONN=Connection*Operative_Level;
      | TLC_SERVICE=TLC_services*Operative_Level;
      | CYBER_FAULT=Cyber_Fault*Operative_Level;
      | MECH_FAULT=Mechanical_Fault;
      mask prompts: Parameter1 "entity name"; Parameter2 "sampling time"; Parameter3 "project"; resources "input resources and state variables"; Parameter10 "Bring state variables to output"; codeupdate "update code from mask"
      mask help: This is a level-2 MATLAB file S-function which demonstrates CISIA entity
      mask DialogControl Container1 Prompt: All parameters
      mask Display: image('Icons/Pipe.png')
  Pipe_Oper2 (413) : M-S-Function  FunctionName=cisia_msfun  Parameters=Parameter1, Parameter2, Parameter3, resources, Parameter10, codeupdate, step_received, step_computed, dynamic_computed, step_sended, id_entity, id_project, id_type, name_type, color  mask(S-function:msfcn_unit_delay){Parameter1='Pipe_Oper2', Parameter2=1, Parameter3='ORO', resources=, Parameter10=off, codeupdate=off, step_received=|, step_computed=, dynamic_computed=, step_sended=|, id_entity=413, id_project=6, id_type=84, name_type=Optical_Wire, color=#99CCFF}
      mask step_received=|
      | Connection=TLC_CONN;
      | TLC_services=TLC_SERVICE;
      | Cyber_Fault=CYBER_FAULT;
      |
      | Mechanical_Fault=max([Mechanical_Fault MECH_FAULT Mechanical_Fault_init]);
      |
      |
      | Operative_Level=1-Mechanical_Fault;
      mask step_sended=|
      | TLC_CONN=Connection*Operative_Level;
      | TLC_SERVICE=TLC_services*Operative_Level;
      | CYBER_FAULT=Cyber_Fault*Operative_Level;
      | MECH_FAULT=Mechanical_Fault;
      mask prompts: Parameter1 "entity name"; Parameter2 "sampling time"; Parameter3 "project"; resources "input resources and state variables"; Parameter10 "Bring state variables to output"; codeupdate "update code from mask"
      mask help: This is a level-2 MATLAB file S-function which demonstrates CISIA entity
      mask DialogControl Container1 Prompt: All parameters
      mask Display: image('Icons/Pipe.png')
  Pipe_Ward (405) : M-S-Function  FunctionName=cisia_msfun  Parameters=Parameter1, Parameter2, Parameter3, resources, Parameter10, codeupdate, step_received, step_computed, dynamic_computed, step_sended, id_entity, id_project, id_type, name_type, color  mask(S-function:msfcn_unit_delay){Parameter1='Pipe_Ward', Parameter2=1, Parameter3='ORO', resources=, Parameter10=off, codeupdate=off, step_received=|, step_computed=, dynamic_computed=, step_sended=|, id_entity=405, id_project=6, id_type=84, name_type=Optical_Wire, color=#99CCFF}
      mask step_received=|
      | Connection=TLC_CONN;
      | TLC_services=TLC_SERVICE;
      | Cyber_Fault=CYBER_FAULT;
      |
      | Mechanical_Fault=max([Mechanical_Fault MECH_FAULT Mechanical_Fault_init]);
      |
      |
      | Operative_Level=1-Mechanical_Fault;
      mask step_sended=|
      | TLC_CONN=Connection*Operative_Level;
      | TLC_SERVICE=TLC_services*Operative_Level;
      | CYBER_FAULT=Cyber_Fault*Operative_Level;
      | MECH_FAULT=Mechanical_Fault;
      mask prompts: Parameter1 "entity name"; Parameter2 "sampling time"; Parameter3 "project"; resources "input resources and state variables"; Parameter10 "Bring state variables to output"; codeupdate "update code from mask"
      mask help: This is a level-2 MATLAB file S-function which demonstrates CISIA entity
      mask DialogControl Container1 Prompt: All parameters
      mask Display: image('Icons/Pipe.png')
  Room_9 (424) : M-S-Function  FunctionName=cisia_msfun  Parameters=Parameter1, Parameter2, Parameter3, resources, Parameter10, codeupdate, step_received, step_computed, dynamic_computed, step_sended, id_entity, id_project, id_type, name_type, color  mask(S-function:msfcn_unit_delay){Parameter1='Room_9', Parameter2=1, Parameter3='ORO', resources=, Parameter10=off, codeupdate=off, step_received=|, step_computed=, dynamic_computed=, step_sended=|, id_entity=424, id_project=6, id_type=9, name_type=Optical_Wire, color=#99CCFF}
      mask step_received=|
      | Connection=TLC_CONN;
      | TLC_services=TLC_SERVICE;
      | Cyber_Fault=CYBER_FAULT;
      |
      | Mechanical_Fault=max([Mechanical_Fault MECH_FAULT Mechanical_Fault_init]);
      |
      |
      | Operative_Level=1-Mechanical_Fault;
      mask step_sended=|
      | TLC_CONN=Connection*Operative_Level;
      | TLC_SERVICE=TLC_services*Operative_Level;
      | CYBER_FAULT=Cyber_Fault*Operative_Level;
      | MECH_FAULT=Mechanical_Fault;
      mask prompts: Parameter1 "entity name"; Parameter2 "sampling time"; Parameter3 "project"; resources "input resources and state variables"; Parameter10 "Bring state variables to output"; codeupdate "update code from mask"
      mask help: This is a level-2 MATLAB file S-function which demonstrates CISIA entity
      mask DialogControl Container1 Prompt: All parameters
      mask Display: image('Icons/Room.png')
  SAVE_13 (13) : M-S-Function  FunctionName=cisia_msfun  Parameters=Parameter1, Parameter2, Parameter3  mask(S-function:msfcn_unit_delay){Parameter1='SAVE_13', Parameter2=1, Parameter3='ORO'}
      mask prompts: Parameter1 "entity name"; Parameter2 "sampling time"; Parameter3 "project"
      mask help: This is a level-2 MATLAB file S-function which demonstrates CISIA entity
      mask Display: disp('SAVE')
  SAVE_14 (14) : M-S-Function  FunctionName=cisia_msfun  Parameters=Parameter1, Parameter2, Parameter3  mask(S-function:msfcn_unit_delay){Parameter1='SAVE_14', Parameter2=1, Parameter3='ORO'}
      mask prompts: Parameter1 "entity name"; Parameter2 "sampling time"; Parameter3 "project"
      mask help: This is a level-2 MATLAB file S-function which demonstrates CISIA entity
      mask Display: disp('SAVE')
  SAVE_15 (15) : M-S-Function  FunctionName=cisia_msfun  Parameters=Parameter1, Parameter2, Parameter3  mask(S-function:msfcn_unit_delay){Parameter1='SAVE_15', Parameter2=1, Parameter3='ORO'}
      mask prompts: Parameter1 "entity name"; Parameter2 "sampling time"; Parameter3 "project"
      mask help: This is a level-2 MATLAB file S-function which demonstrates CISIA entity
      mask Display: disp('SAVE')
  SAVE_16 (16) : M-S-Function  FunctionName=cisia_msfun  Parameters=Parameter1, Parameter2, Parameter3  mask(S-function:msfcn_unit_delay){Parameter1='SAVE_16', Parameter2=1, Parameter3='ORO'}
      mask prompts: Parameter1 "entity name"; Parameter2 "sampling time"; Parameter3 "project"
      mask help: This is a level-2 MATLAB file S-function which demonstrates CISIA entity
      mask Display: disp('SAVE')
  SAVE_17 (17) : M-S-Function  FunctionName=cisia_msfun  Parameters=Parameter1, Parameter2, Parameter3  mask(S-function:msfcn_unit_delay){Parameter1='SAVE_17', Parameter2=1, Parameter3='ORO'}
      mask prompts: Parameter1 "entity name"; Parameter2 "sampling time"; Parameter3 "project"
      mask help: This is a level-2 MATLAB file S-function which demonstrates CISIA entity
      mask Display: disp('SAVE')
  Staff_Room (387) : M-S-Function  FunctionName=cisia_msfun  Parameters=Parameter1, Parameter2, Parameter3, resources, Parameter10, codeupdate, step_received, step_computed, dynamic_computed, step_sended, id_entity, id_project, id_type, name_type, color  mask(S-function:msfcn_unit_delay){Parameter1='Staff_Room', Parameter2=1, Parameter3='ORO', resources=, Parameter10=off, codeupdate=off, step_received=|, step_computed=, dynamic_computed=, step_sended=|, id_entity=387, id_project=6, id_type=26, name_type=Optical_Wire, color=#99CCFF}
      mask step_received=|
      | Connection=TLC_CONN;
      | TLC_services=TLC_SERVICE;
      | Cyber_Fault=CYBER_FAULT;
      |
      | Mechanical_Fault=max([Mechanical_Fault MECH_FAULT Mechanical_Fault_init]);
      |
      |
      | Operative_Level=1-Mechanical_Fault;
      mask step_sended=|
      | TLC_CONN=Connection*Operative_Level;
      | TLC_SERVICE=TLC_services*Operative_Level;
      | CYBER_FAULT=Cyber_Fault*Operative_Level;
      | MECH_FAULT=Mechanical_Fault;
      mask prompts: Parameter1 "entity name"; Parameter2 "sampling time"; Parameter3 "project"; resources "input resources and state variables"; Parameter10 "Bring state variables to output"; codeupdate "update code from mask"
      mask help: This is a level-2 MATLAB file S-function which demonstrates CISIA entity
      mask DialogControl Container1 Prompt: All parameters
      mask Display: disp('Ordinary_Room')
  Subsystem : Subsystem
  Surgery (383) : M-S-Function  FunctionName=cisia_msfun  Parameters=Parameter1, Parameter2, Parameter3, resources, Parameter10, codeupdate, step_received, step_computed, dynamic_computed, step_sended, id_entity, id_project, id_type, name_type, color  mask(S-function:msfcn_unit_delay){Parameter1='Surgery', Parameter2=1, Parameter3='ORO', resources=, Parameter10=off, codeupdate=off, step_received=|, step_computed=, dynamic_computed=, step_sended=|, id_entity=383, id_project=6, id_type=26, name_type=Optical_Wire, color=#99CCFF}
      mask step_received=|
      | Connection=TLC_CONN;
      | TLC_services=TLC_SERVICE;
      | Cyber_Fault=CYBER_FAULT;
      |
      | Mechanical_Fault=max([Mechanical_Fault MECH_FAULT Mechanical_Fault_init]);
      |
      |
      | Operative_Level=1-Mechanical_Fault;
      mask step_sended=|
      | TLC_CONN=Connection*Operative_Level;
      | TLC_SERVICE=TLC_services*Operative_Level;
      | CYBER_FAULT=Cyber_Fault*Operative_Level;
      | MECH_FAULT=Mechanical_Fault;
      mask prompts: Parameter1 "entity name"; Parameter2 "sampling time"; Parameter3 "project"; resources "input resources and state variables"; Parameter10 "Bring state variables to output"; codeupdate "update code from mask"
      mask help: This is a level-2 MATLAB file S-function which demonstrates CISIA entity
      mask DialogControl Container1 Prompt: All parameters
      mask Display: disp('Ordinary_Room')
  Tap (423) : M-S-Function  FunctionName=cisia_msfun  Parameters=Parameter1, Parameter2, Parameter3, resources, Parameter10, codeupdate, step_received, step_computed, dynamic_computed, step_sended, id_entity, id_project, id_type, name_type, color  mask(S-function:msfcn_unit_delay){Parameter1='Tap', Parameter2=1, Parameter3='ORO', resources=, Parameter10=off, codeupdate=off, step_received=|, step_computed=, dynamic_computed=, step_sended=|, id_entity=423, id_project=6, id_type=30, name_type=Optical_Wire, color=#99CCFF}
      mask step_received=|
      | Connection=TLC_CONN;
      | TLC_services=TLC_SERVICE;
      | Cyber_Fault=CYBER_FAULT;
      |
      | Mechanical_Fault=max([Mechanical_Fault MECH_FAULT Mechanical_Fault_init]);
      |
      |
      | Operative_Level=1-Mechanical_Fault;
      mask step_sended=|
      | TLC_CONN=Connection*Operative_Level;
      | TLC_SERVICE=TLC_services*Operative_Level;
      | CYBER_FAULT=Cyber_Fault*Operative_Level;
      | MECH_FAULT=Mechanical_Fault;
      mask prompts: Parameter1 "entity name"; Parameter2 "sampling time"; Parameter3 "project"; resources "input resources and state variables"; Parameter10 "Bring state variables to output"; codeupdate "update code from mask"
      mask help: This is a level-2 MATLAB file S-function which demonstrates CISIA entity
      mask DialogControl Container1 Prompt: All parameters
      mask Display: disp('Tap')
  Terminator : Terminator
  Visit_Room (388) : M-S-Function  FunctionName=cisia_msfun  Parameters=Parameter1, Parameter2, Parameter3, resources, Parameter10, codeupdate, step_received, step_computed, dynamic_computed, step_sended, id_entity, id_project, id_type, name_type, color  mask(S-function:msfcn_unit_delay){Parameter1='Visit_Room', Parameter2=1, Parameter3='ORO', resources=, Parameter10=off, codeupdate=off, step_received=|, step_computed=, dynamic_computed=, step_sended=|, id_entity=388, id_project=6, id_type=26, name_type=Optical_Wire, color=#99CCFF}
      mask step_received=|
      | Connection=TLC_CONN;
      | TLC_services=TLC_SERVICE;
      | Cyber_Fault=CYBER_FAULT;
      |
      | Mechanical_Fault=max([Mechanical_Fault MECH_FAULT Mechanical_Fault_init]);
      |
      |
      | Operative_Level=1-Mechanical_Fault;
      mask step_sended=|
      | TLC_CONN=Connection*Operative_Level;
      | TLC_SERVICE=TLC_services*Operative_Level;
      | CYBER_FAULT=Cyber_Fault*Operative_Level;
      | MECH_FAULT=Mechanical_Fault;
      mask prompts: Parameter1 "entity name"; Parameter2 "sampling time"; Parameter3 "project"; resources "input resources and state variables"; Parameter10 "Bring state variables to output"; codeupdate "update code from mask"
      mask help: This is a level-2 MATLAB file S-function which demonstrates CISIA entity
      mask DialogControl Container1 Prompt: All parameters
      mask Display: disp('Ordinary_Room')
  Waiting_Room (384) : M-S-Function  FunctionName=cisia_msfun  Parameters=Parameter1, Parameter2, Parameter3, resources, Parameter10, codeupdate, step_received, step_computed, dynamic_computed, step_sended, id_entity, id_project, id_type, name_type, color  mask(S-function:msfcn_unit_delay){Parameter1='Waiting_Room', Parameter2=1, Parameter3='ORO', resources=, Parameter10=off, codeupdate=off, step_received=|, step_computed=, dynamic_computed=, step_sended=|, id_entity=384, id_project=6, id_type=26, name_type=Optical_Wire, color=#99CCFF}
      mask step_received=|
      | Connection=TLC_CONN;
      | TLC_services=TLC_SERVICE;
      | Cyber_Fault=CYBER_FAULT;
      |
      | Mechanical_Fault=max([Mechanical_Fault MECH_FAULT Mechanical_Fault_init]);
      |
      |
      | Operative_Level=1-Mechanical_Fault;
      mask step_sended=|
      | TLC_CONN=Connection*Operative_Level;
      | TLC_SERVICE=TLC_services*Operative_Level;
      | CYBER_FAULT=Cyber_Fault*Operative_Level;
      | MECH_FAULT=Mechanical_Fault;
      mask prompts: Parameter1 "entity name"; Parameter2 "sampling time"; Parameter3 "project"; resources "input resources and state variables"; Parameter10 "Bring state variables to output"; codeupdate "update code from mask"
      mask help: This is a level-2 MATLAB file S-function which demonstrates CISIA entity
      mask DialogControl Container1 Prompt: All parameters
      mask Display: disp('Ordinary_Room')
  Wire_MR_1 (370) : M-S-Function  FunctionName=cisia_msfun  Parameters=Parameter1, Parameter2, Parameter3, resources, Parameter10, codeupdate, step_received, step_computed, dynamic_computed, step_sended, id_entity, id_project, id_type, name_type, color  mask(S-function:msfcn_unit_delay){Parameter1='Wire_MR_1', Parameter2=1, Parameter3='ORO', resources=, Parameter10=off, codeupdate=off, step_received=|, step_computed=, dynamic_computed=, step_sended=|, id_entity=370, id_project=6, id_type=29, name_type=Optical_Wire, color=#99CCFF}
      mask step_received=|
      | Connection=TLC_CONN;
      | TLC_services=TLC_SERVICE;
      | Cyber_Fault=CYBER_FAULT;
      |
      | Mechanical_Fault=max([Mechanical_Fault MECH_FAULT Mechanical_Fault_init]);
      |
      |
      | Operative_Level=1-Mechanical_Fault;
      mask step_sended=|
      | TLC_CONN=Connection*Operative_Level;
      | TLC_SERVICE=TLC_services*Operative_Level;
      | CYBER_FAULT=Cyber_Fault*Operative_Level;
      | MECH_FAULT=Mechanical_Fault;
      mask prompts: Parameter1 "entity name"; Parameter2 "sampling time"; Parameter3 "project"; resources "input resources and state variables"; Parameter10 "Bring state variables to output"; codeupdate "update code from mask"
      mask help: This is a level-2 MATLAB file S-function which demonstrates CISIA entity
      mask DialogControl Container1 Prompt: All parameters
      mask Display: disp('Wire_Medical_Room')
  Wire_MR_2 (371) : M-S-Function  FunctionName=cisia_msfun  Parameters=Parameter1, Parameter2, Parameter3, resources, Parameter10, codeupdate, step_received, step_computed, dynamic_computed, step_sended, id_entity, id_project, id_type, name_type, color  mask(S-function:msfcn_unit_delay){Parameter1='Wire_MR_2', Parameter2=1, Parameter3='ORO', resources=, Parameter10=off, codeupdate=off, step_received=|, step_computed=, dynamic_computed=, step_sended=|, id_entity=371, id_project=6, id_type=29, name_type=Optical_Wire, color=#99CCFF}
      mask step_received=|
      | Connection=TLC_CONN;
      | TLC_services=TLC_SERVICE;
      | Cyber_Fault=CYBER_FAULT;
      |
      | Mechanical_Fault=max([Mechanical_Fault MECH_FAULT Mechanical_Fault_init]);
      |
      |
      | Operative_Level=1-Mechanical_Fault;
      mask step_sended=|
      | TLC_CONN=Connection*Operative_Level;
      | TLC_SERVICE=TLC_services*Operative_Level;
      | CYBER_FAULT=Cyber_Fault*Operative_Level;
      | MECH_FAULT=Mechanical_Fault;
      mask prompts: Parameter1 "entity name"; Parameter2 "sampling time"; Parameter3 "project"; resources "input resources and state variables"; Parameter10 "Bring state variables to output"; codeupdate "update code from mask"
      mask help: This is a level-2 MATLAB file S-function which demonstrates CISIA entity
      mask DialogControl Container1 Prompt: All parameters
      mask Display: disp('Wire_Medical_Room')
  Wire_MR_3 (372) : M-S-Function  FunctionName=cisia_msfun  Parameters=Parameter1, Parameter2, Parameter3, resources, Parameter10, codeupdate, step_received, step_computed, dynamic_computed, step_sended, id_entity, id_project, id_type, name_type, color  mask(S-function:msfcn_unit_delay){Parameter1='Wire_MR_3', Parameter2=1, Parameter3='ORO', resources=, Parameter10=off, codeupdate=off, step_received=|, step_computed=, dynamic_computed=, step_sended=|, id_entity=372, id_project=6, id_type=29, name_type=Optical_Wire, color=#99CCFF}
      mask step_received=|
      | Connection=TLC_CONN;
      | TLC_services=TLC_SERVICE;
      | Cyber_Fault=CYBER_FAULT;
      |
      | Mechanical_Fault=max([Mechanical_Fault MECH_FAULT Mechanical_Fault_init]);
      |
      |
      | Operative_Level=1-Mechanical_Fault;
      mask step_sended=|
      | TLC_CONN=Connection*Operative_Level;
      | TLC_SERVICE=TLC_services*Operative_Level;
      | CYBER_FAULT=Cyber_Fault*Operative_Level;
      | MECH_FAULT=Mechanical_Fault;
      mask prompts: Parameter1 "entity name"; Parameter2 "sampling time"; Parameter3 "project"; resources "input resources and state variables"; Parameter10 "Bring state variables to output"; codeupdate "update code from mask"
      mask help: This is a level-2 MATLAB file S-function which demonstrates CISIA entity
      mask DialogControl Container1 Prompt: All parameters
      mask Display: disp('Wire_Medical_Room')
  Wire_MR_4 (373) : M-S-Function  FunctionName=cisia_msfun  Parameters=Parameter1, Parameter2, Parameter3, resources, Parameter10, codeupdate, step_received, step_computed, dynamic_computed, step_sended, id_entity, id_project, id_type, name_type, color  mask(S-function:msfcn_unit_delay){Parameter1='Wire_MR_4', Parameter2=1, Parameter3='ORO', resources=, Parameter10=off, codeupdate=off, step_received=|, step_computed=, dynamic_computed=, step_sended=|, id_entity=373, id_project=6, id_type=29, name_type=Optical_Wire, color=#99CCFF}
      mask step_received=|
      | Connection=TLC_CONN;
      | TLC_services=TLC_SERVICE;
      | Cyber_Fault=CYBER_FAULT;
      |
      | Mechanical_Fault=max([Mechanical_Fault MECH_FAULT Mechanical_Fault_init]);
      |
      |
      | Operative_Level=1-Mechanical_Fault;
      mask step_sended=|
      | TLC_CONN=Connection*Operative_Level;
      | TLC_SERVICE=TLC_services*Operative_Level;
      | CYBER_FAULT=Cyber_Fault*Operative_Level;
      | MECH_FAULT=Mechanical_Fault;
      mask prompts: Parameter1 "entity name"; Parameter2 "sampling time"; Parameter3 "project"; resources "input resources and state variables"; Parameter10 "Bring state variables to output"; codeupdate "update code from mask"
      mask help: This is a level-2 MATLAB file S-function which demonstrates CISIA entity
      mask DialogControl Container1 Prompt: All parameters
      mask Display: disp('Wire_Medical_Room')
  Wire_MR_5 (374) : M-S-Function  FunctionName=cisia_msfun  Parameters=Parameter1, Parameter2, Parameter3, resources, Parameter10, codeupdate, step_received, step_computed, dynamic_computed, step_sended, id_entity, id_project, id_type, name_type, color  mask(S-function:msfcn_unit_delay){Parameter1='Wire_MR_5', Parameter2=1, Parameter3='ORO', resources=, Parameter10=off, codeupdate=off, step_received=|, step_computed=, dynamic_computed=, step_sended=|, id_entity=374, id_project=6, id_type=29, name_type=Optical_Wire, color=#99CCFF}
      mask step_received=|
      | Connection=TLC_CONN;
      | TLC_services=TLC_SERVICE;
      | Cyber_Fault=CYBER_FAULT;
      |
      | Mechanical_Fault=max([Mechanical_Fault MECH_FAULT Mechanical_Fault_init]);
      |
      |
      | Operative_Level=1-Mechanical_Fault;
      mask step_sended=|
      | TLC_CONN=Connection*Operative_Level;
      | TLC_SERVICE=TLC_services*Operative_Level;
      | CYBER_FAULT=Cyber_Fault*Operative_Level;
      | MECH_FAULT=Mechanical_Fault;
      mask prompts: Parameter1 "entity name"; Parameter2 "sampling time"; Parameter3 "project"; resources "input resources and state variables"; Parameter10 "Bring state variables to output"; codeupdate "update code from mask"
      mask help: This is a level-2 MATLAB file S-function which demonstrates CISIA entity
      mask DialogControl Container1 Prompt: All parameters
      mask Display: disp('Wire_Medical_Room')
  Wire_MR_6 (375) : M-S-Function  FunctionName=cisia_msfun  Parameters=Parameter1, Parameter2, Parameter3, resources, Parameter10, codeupdate, step_received, step_computed, dynamic_computed, step_sended, id_entity, id_project, id_type, name_type, color  mask(S-function:msfcn_unit_delay){Parameter1='Wire_MR_6', Parameter2=1, Parameter3='ORO', resources=, Parameter10=off, codeupdate=off, step_received=|, step_computed=, dynamic_computed=, step_sended=|, id_entity=375, id_project=6, id_type=29, name_type=Optical_Wire, color=#99CCFF}
      mask step_received=|
      | Connection=TLC_CONN;
      | TLC_services=TLC_SERVICE;
      | Cyber_Fault=CYBER_FAULT;
      |
      | Mechanical_Fault=max([Mechanical_Fault MECH_FAULT Mechanical_Fault_init]);
      |
      |
      | Operative_Level=1-Mechanical_Fault;
      mask step_sended=|
      | TLC_CONN=Connection*Operative_Level;
      | TLC_SERVICE=TLC_services*Operative_Level;
      | CYBER_FAULT=Cyber_Fault*Operative_Level;
      | MECH_FAULT=Mechanical_Fault;
      mask prompts: Parameter1 "entity name"; Parameter2 "sampling time"; Parameter3 "project"; resources "input resources and state variables"; Parameter10 "Bring state variables to output"; codeupdate "update code from mask"
      mask help: This is a level-2 MATLAB file S-function which demonstrates CISIA entity
      mask DialogControl Container1 Prompt: All parameters
      mask Display: disp('Wire_Medical_Room')
  Wire_OP_1 (376) : M-S-Function  FunctionName=cisia_msfun  Parameters=Parameter1, Parameter2, Parameter3, resources, Parameter10, codeupdate, step_received, step_computed, dynamic_computed, step_sended, id_entity, id_project, id_type, name_type, color  mask(S-function:msfcn_unit_delay){Parameter1='Wire_OP_1', Parameter2=1, Parameter3='ORO', resources=, Parameter10=off, codeupdate=off, step_received=|, step_computed=, dynamic_computed=, step_sended=|, id_entity=376, id_project=6, id_type=29, name_type=Optical_Wire, color=#99CCFF}
      mask step_received=|
      | Connection=TLC_CONN;
      | TLC_services=TLC_SERVICE;
      | Cyber_Fault=CYBER_FAULT;
      |
      | Mechanical_Fault=max([Mechanical_Fault MECH_FAULT Mechanical_Fault_init]);
      |
      |
      | Operative_Level=1-Mechanical_Fault;
      mask step_sended=|
      | TLC_CONN=Connection*Operative_Level;
      | TLC_SERVICE=TLC_services*Operative_Level;
      | CYBER_FAULT=Cyber_Fault*Operative_Level;
      | MECH_FAULT=Mechanical_Fault;
      mask prompts: Parameter1 "entity name"; Parameter2 "sampling time"; Parameter3 "project"; resources "input resources and state variables"; Parameter10 "Bring state variables to output"; codeupdate "update code from mask"
      mask help: This is a level-2 MATLAB file S-function which demonstrates CISIA entity
      mask DialogControl Container1 Prompt: All parameters
      mask Display: disp('Wire_Medical_Room')
  Wire_OP_2 (377) : M-S-Function  FunctionName=cisia_msfun  Parameters=Parameter1, Parameter2, Parameter3, resources, Parameter10, codeupdate, step_received, step_computed, dynamic_computed, step_sended, id_entity, id_project, id_type, name_type, color  mask(S-function:msfcn_unit_delay){Parameter1='Wire_OP_2', Parameter2=1, Parameter3='ORO', resources=, Parameter10=off, codeupdate=off, step_received=|, step_computed=, dynamic_computed=, step_sended=|, id_entity=377, id_project=6, id_type=29, name_type=Optical_Wire, color=#99CCFF}
      mask step_received=|
      | Connection=TLC_CONN;
      | TLC_services=TLC_SERVICE;
      | Cyber_Fault=CYBER_FAULT;
      |
      | Mechanical_Fault=max([Mechanical_Fault MECH_FAULT Mechanical_Fault_init]);
      |
      |
      | Operative_Level=1-Mechanical_Fault;
      mask step_sended=|
      | TLC_CONN=Connection*Operative_Level;
      | TLC_SERVICE=TLC_services*Operative_Level;
      | CYBER_FAULT=Cyber_Fault*Operative_Level;
      | MECH_FAULT=Mechanical_Fault;
      mask prompts: Parameter1 "entity name"; Parameter2 "sampling time"; Parameter3 "project"; resources "input resources and state variables"; Parameter10 "Bring state variables to output"; codeupdate "update code from mask"
      mask help: This is a level-2 MATLAB file S-function which demonstrates CISIA entity
      mask DialogControl Container1 Prompt: All parameters
      mask Display: disp('Wire_Medical_Room')
  Wire_OR_1 (378) : M-S-Function  FunctionName=cisia_msfun  Parameters=Parameter1, Parameter2, Parameter3, resources, Parameter10, codeupdate, step_received, step_computed, dynamic_computed, step_sended, id_entity, id_project, id_type, name_type, color  mask(S-function:msfcn_unit_delay){Parameter1='Wire_OR_1', Parameter2=1, Parameter3='ORO', resources=, Parameter10=off, codeupdate=off, step_received=|, step_computed=, dynamic_computed=, step_sended=|, id_entity=378, id_project=6, id_type=29, name_type=Optical_Wire, color=#99CCFF}
      mask step_received=|
      | Connection=TLC_CONN;
      | TLC_services=TLC_SERVICE;
      | Cyber_Fault=CYBER_FAULT;
      |
      | Mechanical_Fault=max([Mechanical_Fault MECH_FAULT Mechanical_Fault_init]);
      |
      |
      | Operative_Level=1-Mechanical_Fault;
      mask step_sended=|
      | TLC_CONN=Connection*Operative_Level;
      | TLC_SERVICE=TLC_services*Operative_Level;
      | CYBER_FAULT=Cyber_Fault*Operative_Level;
      | MECH_FAULT=Mechanical_Fault;
      mask prompts: Parameter1 "entity name"; Parameter2 "sampling time"; Parameter3 "project"; resources "input resources and state variables"; Parameter10 "Bring state variables to output"; codeupdate "update code from mask"
      mask help: This is a level-2 MATLAB file S-function which demonstrates CISIA entity
      mask DialogControl Container1 Prompt: All parameters
      mask Display: disp('Wire_Medical_Room')
  Wire_OR_2 (379) : M-S-Function  FunctionName=cisia_msfun  Parameters=Parameter1, Parameter2, Parameter3, resources, Parameter10, codeupdate, step_received, step_computed, dynamic_computed, step_sended, id_entity, id_project, id_type, name_type, color  mask(S-function:msfcn_unit_delay){Parameter1='Wire_OR_2', Parameter2=1, Parameter3='ORO', resources=, Parameter10=off, codeupdate=off, step_received=|, step_computed=, dynamic_computed=, step_sended=|, id_entity=379, id_project=6, id_type=29, name_type=Optical_Wire, color=#99CCFF}
      mask step_received=|
      | Connection=TLC_CONN;
      | TLC_services=TLC_SERVICE;
      | Cyber_Fault=CYBER_FAULT;
      |
      | Mechanical_Fault=max([Mechanical_Fault MECH_FAULT Mechanical_Fault_init]);
      |
      |
      | Operative_Level=1-Mechanical_Fault;
      mask step_sended=|
      | TLC_CONN=Connection*Operative_Level;
      | TLC_SERVICE=TLC_services*Operative_Level;
      | CYBER_FAULT=Cyber_Fault*Operative_Level;
      | MECH_FAULT=Mechanical_Fault;
      mask prompts: Parameter1 "entity name"; Parameter2 "sampling time"; Parameter3 "project"; resources "input resources and state variables"; Parameter10 "Bring state variables to output"; codeupdate "update code from mask"
      mask help: This is a level-2 MATLAB file S-function which demonstrates CISIA entity
      mask DialogControl Container1 Prompt: All parameters
      mask Display: disp('Wire_Medical_Room')
  Wire_OR_3 (380) : M-S-Function  FunctionName=cisia_msfun  Parameters=Parameter1, Parameter2, Parameter3, resources, Parameter10, codeupdate, step_received, step_computed, dynamic_computed, step_sended, id_entity, id_project, id_type, name_type, color  mask(S-function:msfcn_unit_delay){Parameter1='Wire_OR_3', Parameter2=1, Parameter3='ORO', resources=, Parameter10=off, codeupdate=off, step_received=|, step_computed=, dynamic_computed=, step_sended=|, id_entity=380, id_project=6, id_type=29, name_type=Optical_Wire, color=#99CCFF}
      mask step_received=|
      | Connection=TLC_CONN;
      | TLC_services=TLC_SERVICE;
      | Cyber_Fault=CYBER_FAULT;
      |
      | Mechanical_Fault=max([Mechanical_Fault MECH_FAULT Mechanical_Fault_init]);
      |
      |
      | Operative_Level=1-Mechanical_Fault;
      mask step_sended=|
      | TLC_CONN=Connection*Operative_Level;
      | TLC_SERVICE=TLC_services*Operative_Level;
      | CYBER_FAULT=Cyber_Fault*Operative_Level;
      | MECH_FAULT=Mechanical_Fault;
      mask prompts: Parameter1 "entity name"; Parameter2 "sampling time"; Parameter3 "project"; resources "input resources and state variables"; Parameter10 "Bring state variables to output"; codeupdate "update code from mask"
      mask help: This is a level-2 MATLAB file S-function which demonstrates CISIA entity
      mask DialogControl Container1 Prompt: All parameters
      mask Display: disp('Wire_Medical_Room')
  Wire_S_1 (381) : M-S-Function  FunctionName=cisia_msfun  Parameters=Parameter1, Parameter2, Parameter3, resources, Parameter10, codeupdate, step_received, step_computed, dynamic_computed, step_sended, id_entity, id_project, id_type, name_type, color  mask(S-function:msfcn_unit_delay){Parameter1='Wire_S_1', Parameter2=1, Parameter3='ORO', resources=, Parameter10=off, codeupdate=off, step_received=|, step_computed=, dynamic_computed=, step_sended=|, id_entity=381, id_project=6, id_type=29, name_type=Optical_Wire, color=#99CCFF}
      mask step_received=|
      | Connection=TLC_CONN;
      | TLC_services=TLC_SERVICE;
      | Cyber_Fault=CYBER_FAULT;
      |
      | Mechanical_Fault=max([Mechanical_Fault MECH_FAULT Mechanical_Fault_init]);
      |
      |
      | Operative_Level=1-Mechanical_Fault;
      mask step_sended=|
      | TLC_CONN=Connection*Operative_Level;
      | TLC_SERVICE=TLC_services*Operative_Level;
      | CYBER_FAULT=Cyber_Fault*Operative_Level;
      | MECH_FAULT=Mechanical_Fault;
      mask prompts: Parameter1 "entity name"; Parameter2 "sampling time"; Parameter3 "project"; resources "input resources and state variables"; Parameter10 "Bring state variables to output"; codeupdate "update code from mask"
      mask help: This is a level-2 MATLAB file S-function which demonstrates CISIA entity
      mask DialogControl Container1 Prompt: All parameters
      mask Display: disp('Wire_Medical_Room')
  Wire_S_2 (382) : M-S-Function  FunctionName=cisia_msfun  Parameters=Parameter1, Parameter2, Parameter3, resources, Parameter10, codeupdate, step_received, step_computed, dynamic_computed, step_sended, id_entity, id_project, id_type, name_type, color  mask(S-function:msfcn_unit_delay){Parameter1='Wire_S_2', Parameter2=1, Parameter3='ORO', resources=, Parameter10=off, codeupdate=off, step_received=|, step_computed=, dynamic_computed=, step_sended=|, id_entity=382, id_project=6, id_type=29, name_type=Optical_Wire, color=#99CCFF}
      mask step_received=|
      | Connection=TLC_CONN;
      | TLC_services=TLC_SERVICE;
      | Cyber_Fault=CYBER_FAULT;
      |
      | Mechanical_Fault=max([Mechanical_Fault MECH_FAULT Mechanical_Fault_init]);
      |
      |
      | Operative_Level=1-Mechanical_Fault;
      mask step_sended=|
      | TLC_CONN=Connection*Operative_Level;
      | TLC_SERVICE=TLC_services*Operative_Level;
      | CYBER_FAULT=Cyber_Fault*Operative_Level;
      | MECH_FAULT=Mechanical_Fault;
      mask prompts: Parameter1 "entity name"; Parameter2 "sampling time"; Parameter3 "project"; resources "input resources and state variables"; Parameter10 "Bring state variables to output"; codeupdate "update code from mask"
      mask help: This is a level-2 MATLAB file S-function which demonstrates CISIA entity
      mask DialogControl Container1 Prompt: All parameters
      mask Display: disp('Wire_Medical_Room')
  wires:
  Wire_OP_1 (376)/1 -> Operating_1 (403)/4  "POWER"
  Humidifier (394)/1 -> Cooling_Coil (395)/2  "AIR"
  Heating_Coil (393)/1 -> Humidifier (394)/2  "AIR"
  Tap (423)/1 -> Pipe_1 (335)/1  "WATER"
  Wire_OR_3 (380)/1 -> Drug_Store (389)/1, Equipment_Warehouse (390)/1  "POWER"
  Wire_MR_4 (373)/1 -> Medical_4 (400)/4  "POWER"
  Duct_2 (367)/1 -> Medical_3 (399)/6, Medical_4 (400)/6, Waiting_Room (384)/2, Surgery (383)/2, Doctor_Room (414)/2  "AIR"
  Pipe_Oper2 (413)/2 -> Mux4/8  "PIPE_QoS"
  Fan (391)/1 -> Heating_Coil (393)/2  "AIR"
  Pipe_Oper1 (412)/1 -> Operating_1 (403)/5  "WATER"
  Pipe_Medical3 (408)/1 -> Medical_3 (399)/5  "WATER"
  Pipe_Oper2 (413)/1 -> Operating_2 (404)/5  "WATER"
  Wire_MR_5 (374)/1 -> Medical_5 (401)/4  "POWER"
  Wire_MR_3 (372)/1 -> Medical_3 (399)/4  "POWER"
  Pipe_Oper1 (412)/2 -> Mux4/7  "PIPE_QoS"
  Wire_MR_3 (372)/2 -> Mux1/10  "WIRE_QoS"
  Pipe_Medical4 (409)/1 -> Medical_4 (400)/5  "WATER"
  Pipe_Medical5 (410)/2 -> Mux4/5  "PIPE_QoS"
  Mux3/1 -> AIR_QoS/1
  Pipe_Medical6 (411)/2 -> Mux4/6  "PIPE_QoS"
  Pipe_Medical2 (407)/2 -> Mux4/3  "PIPE_QoS"
  Pipe_Medical6 (411)/1 -> Medical_6 (402)/5  "WATER"
  Wire_MR_4 (373)/2 -> Mux1/5  "WIRE_QoS"
  Duct_4 (369)/2 -> Mux3/3  "DUCT_QoS"
  Pipe_1 (335)/2 -> Mux4/9  "PIPE_QoS"
  Pipe_Medical4 (409)/2 -> Mux4/4  "PIPE_QoS"
  Wire_S_1 (381)/2 -> Mux1/1  "WIRE_QoS"
  Wire_S_1 (381)/1 -> Oxygen_Pump (426)/1, Fan (391)/1, Humidifier (394)/1, Cooling_Coil (395)/1, Heating_Coil (393)/1  "POWER"
  Duct_3 (368)/2 -> Mux3/1  "DUCT_QoS"
  Duct_2 (367)/2 -> Mux3/2  "DUCT_QoS"
  Pipe_Medical5 (410)/1 -> Medical_5 (401)/5  "WATER"
  Cooling_Coil (395)/1 -> Duct_4 (369)/1, Duct_3 (368)/1, Duct_2 (367)/1, Duct_1 (366)/1  "AIR"
  Duct_3 (368)/1 -> Medical_2 (398)/6, Visit_Room (388)/2, Staff_Room (387)/2, Material_Room (386)/2, Cafeteria (385)/2  "AIR"
  Pipe_Medical3 (408)/2 -> Mux4/2  "PIPE_QoS"
  Duct_4 (369)/1 -> Medical_6 (402)/6, Medical_5 (401)/6, Equipment_Warehouse (390)/2, Drug_Store (389)/2  "AIR"
  Pipe_Ward (405)/2 -> Mux4/10  "PIPE_QoS"
  Wire_OR_2 (379)/1 -> Visit_Room (388)/1, Staff_Room (387)/1, Material_Room (386)/1, Cafeteria (385)/1  "POWER"
  Wire_MR_6 (375)/1 -> Medical_6 (402)/4  "POWER"
  Wire_MR_5 (374)/2 -> Mux1/4  "WIRE_QoS"
  Autoclave (425)/1 -> Pipe_Ward (405)/1  "WATER"
  Pipe_Medical2 (407)/1 -> Medical_2 (398)/5  "WATER"
  Pipe_Ward (405)/1 -> Pipe_Medical5 (410)/1, Pipe_Oper2 (413)/1, Pipe_Oper1 (412)/1, Pipe_Medical6 (411)/1, Pipe_Medical4 (409)/1, Pipe_Medical3 (408)/1, Pipe_Medical2 (407)/1, Pipe_Medical1 (406)/1  "WATER"
  Wire_MR_6 (375)/2 -> Mux1/6  "WIRE_QoS"
  Wire_MR_2 (371)/1 -> Medical_2 (398)/4  "POWER"
  Pipe_Medical1 (406)/2 -> Mux4/1  "PIPE_QoS"
  Mux4/1 -> Mean3/1
  Wire_OP_2 (377)/2 -> Mux1/7  "WIRE_QoS"
  Wire_OR_1 (378)/2 -> Mux1/9  "WIRE_QoS"
  Mux1/1 -> POWER_QoS/1
  Wire_MR_1 (370)/2 -> Mux1/12  "WIRE_QoS"
  Wire_OR_1 (378)/1 -> Waiting_Room (384)/1, Surgery (383)/1, Doctor_Room (414)/1  "POWER"
  Wire_OR_2 (379)/2 -> Mux1/3  "WIRE_QoS"
  Wire_MR_2 (371)/2 -> Mux1/11  "WIRE_QoS"
  Wire_OR_3 (380)/2 -> Mux1/2  "WIRE_QoS"
  Duct_1 (366)/1 -> Operating_2 (404)/6, Operating_1 (403)/6, Medical_1 (397)/6  "AIR"
  Wire_OP_2 (377)/1 -> Operating_2 (404)/4  "POWER"
  Duct_1 (366)/2 -> Mux3/4  "DUCT_QoS"
  L2S_1 (396)/1 -> BTS_1 (428)/1, Medical_1 (397)/1, Operating_2 (404)/1, Operating_1 (403)/1, Medical_6 (402)/1, Medical_5 (401)/1, Medical_4 (400)/1, Medical_3 (399)/1, Medical_2 (398)/1  "TLC_CONN"
  L2S_1 (396)/2 -> BTS_1 (428)/2, Medical_1 (397)/2, Operating_2 (404)/2, Operating_1 (403)/2, Medical_6 (402)/2, Medical_5 (401)/2, Medical_4 (400)/2, Medical_3 (399)/2, Medical_2 (398)/2  "TLC_SERVICE"
  L2S_1 (396)/3 -> BTS_1 (428)/3, Medical_1 (397)/3, Operating_2 (404)/3, Operating_1 (403)/3, Medical_6 (402)/3, Medical_5 (401)/3, Medical_4 (400)/3, Medical_3 (399)/3, Medical_2 (398)/3  "CYBER_FAULT"
  [MOBILE_QoS] -> Medical_1 (397)/7, Medical_2 (398)/7, Medical_3 (399)/7, Medical_4 (400)/7, Medical_5 (401)/7, Medical_6 (402)/7, Operating_1 (403)/7, Operating_2 (404)/7  "MOBILE_QoS"
  Mean3/1 -> SAVE_13 (13)/1  "PIPE_QoS"
  Staff_Room (387)/1 -> Mux5/6  "ORDINARY_ROOM_QoS"
  AIR_QoS/1 -> SAVE_16 (16)/1
  POWER_QoS/1 -> SAVE_17 (17)/1
  Room_9 (424)/1 -> L2S_1 (396)/5  "ROOM_QoS"
  Doctor_Room (414)/1 -> Mux5/1  "ORDINARY_ROOM_QoS"
  Surgery (383)/1 -> Mux5/2  "ORDINARY_ROOM_QoS"
  Waiting_Room (384)/1 -> Mux5/3  "ORDINARY_ROOM_QoS"
  Cafeteria (385)/1 -> Mux5/4  "ORDINARY_ROOM_QoS"
  Material_Room (386)/1 -> Mux5/5  "ORDINARY_ROOM_QoS"
  Visit_Room (388)/1 -> Mux5/7  "ORDINARY_ROOM_QoS"
  Drug_Store (389)/1 -> Mux5/8  "ORDINARY_ROOM_QoS"
  Equipment_Warehouse (390)/1 -> Mux5/9  "ORDINARY_ROOM_QoS"
  Mux5/1 -> Mean2/1
  Mean2/1 -> SAVE_14 (14)/1  "ORDINARY_ROOM_QoS"
  Operating_2 (404)/1 -> Mux7/8  "MEDICAL_ROOM_QoS"
  Operating_1 (403)/1 -> Mux7/7  "MEDICAL_ROOM_QoS"
  Medical_6 (402)/1 -> Mux7/6  "MEDICAL_ROOM_QoS"
  Medical_5 (401)/1 -> Mux7/5  "MEDICAL_ROOM_QoS"
  Medical_4 (400)/1 -> Mux7/4  "MEDICAL_ROOM_QoS"
  Medical_3 (399)/1 -> Mux7/3  "MEDICAL_ROOM_QoS"
  Medical_2 (398)/1 -> Mux7/2  "MEDICAL_ROOM_QoS"
  Medical_1 (397)/1 -> Mux7/1  "MEDICAL_ROOM_QoS"
  Mux7/1 -> Mean4/1
  Mean4/1 -> SAVE_15 (15)/1  "MEDICAL_ROOM_QoS"
  Oxygen_Pump (426)/1 -> Oxygen_Duct_7 (421)/1, Oxygen_Duct_8 (422)/1, Oxygen_Duct_6 (420)/1, Oxygen_Duct_5 (419)/1, Oxygen_Duct_4 (418)/1, Oxygen_Duct_3 (417)/1, Oxygen_Duct_2 (416)/1, Oxygen_Duct_1 (415)/1  "OXYGEN"
  Oxygen_Duct_2 (416)/1 -> Medical_2 (398)/8  "OXYGEN"
  Oxygen_Duct_3 (417)/1 -> Medical_3 (399)/8  "OXYGEN"
  Oxygen_Duct_4 (418)/1 -> Medical_4 (400)/8  "OXYGEN"
  Oxygen_Duct_5 (419)/1 -> Medical_5 (401)/8  "OXYGEN"
  Oxygen_Duct_6 (420)/1 -> Medical_6 (402)/8  "OXYGEN"
  Oxygen_Duct_7 (421)/1 -> Operating_1 (403)/8  "OXYGEN"
  Oxygen_Duct_8 (422)/1 -> Operating_2 (404)/8  "OXYGEN"
  Wire_OP_1 (376)/2 -> Mux1/8  "WIRE_QoS"
  CISIA_MASTER (0)/4 -> Display21/1  "TIME PAST"
  CISIA_MASTER (0)/1 -> Display18/1  "MINOR HITS"
  CISIA_MASTER (0)/2 -> Display19/1  "MAJOR HITS"
  CISIA_MASTER (0)/3 -> Display20/1  "DELTA TIME"
  Pipe_1 (335)/1 -> Autoclave (425)/2  "WATER"
  Wire_S_2 (382)/1 -> Autoclave (425)/1  "POWER"
  Wire_S_2 (382)/2 -> Mux1/13  "WIRE_QoS"
  Wire_MR_1 (370)/1 -> Medical_1 (397)/4  "POWER"
  Pipe_Medical1 (406)/1 -> Medical_1 (397)/5  "WATER"
  Oxygen_Duct_1 (415)/1 -> Medical_1 (397)/8  "OXYGEN"
  Subsystem/1(TLC_CONN) -> L2S_1 (396)/1  "TLC_CONN"
  Subsystem/2(TLC_SERVICE) -> L2S_1 (396)/2  "TLC_SERVICE"
  Subsystem/3(CYBER_FAULT) -> L2S_1 (396)/3  "CYBER_FAULT"
  ANT_1 (427)/1 -> Mobile_1 (429)/1  "TLC_SERVICE"
  ANT_1 (427)/3 -> Mobile_1 (429)/3  "R_CONN"
  Mobile_1 (429)/1 -> [MOBILE_QoS]  "MOBILE_QoS"
  BTS_1 (428)/2 -> ANT_1 (427)/2  "CYBER_FAULT"
  BTS_1 (428)/1 -> ANT_1 (427)/1  "TLC_SERVICE"
  ANT_1 (427)/2 -> Mobile_1 (429)/2  "CYBER_FAULT"
  Generator (392)/1 -> ANT_1 (427)/3, Wire_S_2 (382)/1, L2S_1 (396)/4, Wire_MR_1 (370)/1, Wire_S_1 (381)/1, Wire_OP_2 (377)/1, Wire_OP_1 (376)/1, Wire_MR_6 (375)/1, Wire_MR_5 (374)/1, Wire_MR_4 (373)/1, Wire_MR_3 (372)/1, Wire_MR_2 (371)/1, Wire_OR_3 (380)/1, Wire_OR_2 (379)/1, Wire_OR_1 (378)/1, Room_9 (424)/1  "POWER"
  BTS_1 (428)/3 -> ANT_1 (427)/4  "BTS_CONN"
  Constant/1 -> Pipe_1 (335)/2, Pipe_Ward (405)/2, Pipe_Oper2 (413)/2, Pipe_Oper1 (412)/2, Pipe_Medical6 (411)/2, Pipe_Medical5 (410)/2, Pipe_Medical4 (409)/2, Pipe_Medical3 (408)/2, Pipe_Medical2 (407)/2, Pipe_Medical1 (406)/2  "VALVE_QoS"
  Constant1/1 -> Pipe_Ward (405)/3, Pipe_Medical2 (407)/3, Pipe_Oper2 (413)/3, Pipe_Oper1 (412)/3, Pipe_Medical6 (411)/3, Pipe_Medical5 (410)/3, Pipe_Medical4 (409)/3, Pipe_Medical3 (408)/3, Pipe_Medical1 (406)/3, Pipe_1 (335)/3  "PUMP_QoS"
  Generator (392)/2 -> Terminator/1  "GENERATOR_QoS"
